simulink model "model_compatible"  (Simulink 7.5)
(part 2 of 2)

  bus2 : powerlib/Measurements/Load Flow Bus  LConnTagsString=a  Phases=single  Connectors=on one side  ID=bus2  Vbase=330000  Vref=1  Vangle=0  VLF=1  VLFb=1  VLFc=1  angleLF=0  angleLFb=0  angleLFc=0
      settings: AttributesFormatString=|
      | %<ID>
      | %<Vbase>V
      | %<VLF>pu
      | %<angleLF>deg.
      | %<Name>
  bus20 : powerlib/Measurements/Load Flow Bus  LConnTagsString=a  Phases=single  Connectors=on one side  ID=bus20  Vbase=330000  Vref=1  Vangle=0  VLF=1  VLFb=1  VLFc=1  angleLF=0  angleLFb=0  angleLFc=0
      settings: AttributesFormatString=|
      | %<ID>
      | %<Vbase>V
      | %<VLF>pu
      | %<angleLF>deg.
      | %<Name>
  bus21 : powerlib/Measurements/Load Flow Bus  LConnTagsString=a  Phases=single  Connectors=on one side  ID=bus21  Vbase=330000  Vref=1  Vangle=0  VLF=1  VLFb=1  VLFc=1  angleLF=0  angleLFb=0  angleLFc=0
      settings: AttributesFormatString=|
      | %<ID>
      | %<Vbase>V
      | %<VLF>pu
      | %<angleLF>deg.
      | %<Name>
  bus22 : powerlib/Measurements/Load Flow Bus  LConnTagsString=a  Phases=single  Connectors=on one side  ID=bus22  Vbase=330000  Vref=1  Vangle=0  VLF=1  VLFb=1  VLFc=1  angleLF=0  angleLFb=0  angleLFc=0
      settings: AttributesFormatString=|
      | %<ID>
      | %<Vbase>V
      | %<VLF>pu
      | %<angleLF>deg.
      | %<Name>
  bus23 : powerlib/Measurements/Load Flow Bus  LConnTagsString=a  Phases=single  Connectors=on one side  ID=bus23  Vbase=330000  Vref=1  Vangle=0  VLF=1  VLFb=1  VLFc=1  angleLF=0  angleLFb=0  angleLFc=0
      settings: AttributesFormatString=|
      | %<ID>
      | %<Vbase>V
      | %<VLF>pu
      | %<angleLF>deg.
      | %<Name>
  bus24 : powerlib/Measurements/Load Flow Bus  LConnTagsString=a  Phases=single  Connectors=on one side  ID=bus24  Vbase=330000  Vref=1  Vangle=0  VLF=1  VLFb=1  VLFc=1  angleLF=0  angleLFb=0  angleLFc=0
      settings: AttributesFormatString=|
      | %<ID>
      | %<Vbase>V
      | %<VLF>pu
      | %<angleLF>deg.
      | %<Name>
  bus25 : powerlib/Measurements/Load Flow Bus  LConnTagsString=a  Phases=single  Connectors=on one side  ID=bus25  Vbase=330000  Vref=1  Vangle=0  VLF=1  VLFb=1  VLFc=1  angleLF=0  angleLFb=0  angleLFc=0
      settings: AttributesFormatString=|
      | %<ID>
      | %<Vbase>V
      | %<VLF>pu
      | %<angleLF>deg.
      | %<Name>
  bus26 : powerlib/Measurements/Load Flow Bus  LConnTagsString=a  Phases=single  Connectors=on one side  ID=bus26  Vbase=330000  Vref=1  Vangle=0  VLF=1  VLFb=1  VLFc=1  angleLF=0  angleLFb=0  angleLFc=0
      settings: AttributesFormatString=|
      | %<ID>
      | %<Vbase>V
      | %<VLF>pu
      | %<angleLF>deg.
      | %<Name>
  bus27 : powerlib/Measurements/Load Flow Bus  LConnTagsString=a  Phases=single  Connectors=on one side  ID=bus27  Vbase=330000  Vref=1  Vangle=0  VLF=1  VLFb=1  VLFc=1  angleLF=0  angleLFb=0  angleLFc=0
      settings: AttributesFormatString=|
      | %<ID>
      | %<Vbase>V
      | %<VLF>pu
      | %<angleLF>deg.
      | %<Name>
  bus28 : powerlib/Measurements/Load Flow Bus  LConnTagsString=a  Phases=single  Connectors=on one side  ID=bus28  Vbase=330000  Vref=1  Vangle=0  VLF=1  VLFb=1  VLFc=1  angleLF=0  angleLFb=0  angleLFc=0
      settings: AttributesFormatString=|
      | %<ID>
      | %<Vbase>V
      | %<VLF>pu
      | %<angleLF>deg.
      | %<Name>
  bus29 : powerlib/Measurements/Load Flow Bus  LConnTagsString=a  Phases=single  Connectors=on one side  ID=bus29  Vbase=330000  Vref=1  Vangle=0  VLF=1  VLFb=1  VLFc=1  angleLF=0  angleLFb=0  angleLFc=0
      settings: AttributesFormatString=|
      | %<ID>
      | %<Vbase>V
      | %<VLF>pu
      | %<angleLF>deg.
      | %<Name>
  bus3 : powerlib/Measurements/Load Flow Bus  LConnTagsString=a  Phases=single  Connectors=on one side  ID=bus3  Vbase=330000  Vref=1  Vangle=0  VLF=1  VLFb=1  VLFc=1  angleLF=0  angleLFb=0  angleLFc=0
      settings: AttributesFormatString=|
      | %<ID>
      | %<Vbase>V
      | %<VLF>pu
      | %<angleLF>deg.
      | %<Name>
  bus30 : powerlib/Measurements/Load Flow Bus  LConnTagsString=a  Phases=single  Connectors=on one side  ID=bus30  Vbase=330000  Vref=1  Vangle=0  VLF=1  VLFb=1  VLFc=1  angleLF=0  angleLFb=0  angleLFc=0
      settings: AttributesFormatString=|
      | %<ID>
      | %<Vbase>V
      | %<VLF>pu
      | %<angleLF>deg.
      | %<Name>
  bus31 : powerlib/Measurements/Load Flow Bus  LConnTagsString=a  Phases=single  Connectors=on one side  ID=bus31  Vbase=330000  Vref=1  Vangle=0  VLF=1  VLFb=1  VLFc=1  angleLF=0  angleLFb=0  angleLFc=0
      settings: AttributesFormatString=|
      | %<ID>
      | %<Vbase>V
      | %<VLF>pu
      | %<angleLF>deg.
      | %<Name>
  bus32 : powerlib/Measurements/Load Flow Bus  LConnTagsString=a  Phases=single  Connectors=on one side  ID=bus32  Vbase=330000  Vref=1  Vangle=0  VLF=1  VLFb=1  VLFc=1  angleLF=0  angleLFb=0  angleLFc=0
      settings: AttributesFormatString=|
      | %<ID>
      | %<Vbase>V
      | %<VLF>pu
      | %<angleLF>deg.
      | %<Name>
  bus33 : powerlib/Measurements/Load Flow Bus  LConnTagsString=a  Phases=single  Connectors=on one side  ID=bus33  Vbase=330000  Vref=1  Vangle=0  VLF=1  VLFb=1  VLFc=1  angleLF=0  angleLFb=0  angleLFc=0
      settings: AttributesFormatString=|
      | %<ID>
      | %<Vbase>V
      | %<VLF>pu
      | %<angleLF>deg.
      | %<Name>
  bus34 : powerlib/Measurements/Load Flow Bus  LConnTagsString=a  Phases=single  Connectors=on one side  ID=bus34  Vbase=330000  Vref=1  Vangle=0  VLF=1  VLFb=1  VLFc=1  angleLF=0  angleLFb=0  angleLFc=0
      settings: AttributesFormatString=|
      | %<ID>
      | %<Vbase>V
      | %<VLF>pu
      | %<angleLF>deg.
      | %<Name>
  bus35 : powerlib/Measurements/Load Flow Bus  LConnTagsString=a  Phases=single  Connectors=on one side  ID=bus35  Vbase=330000  Vref=1  Vangle=0  VLF=1  VLFb=1  VLFc=1  angleLF=0  angleLFb=0  angleLFc=0
      settings: AttributesFormatString=|
      | %<ID>
      | %<Vbase>V
      | %<VLF>pu
      | %<angleLF>deg.
      | %<Name>
  bus36 : powerlib/Measurements/Load Flow Bus  LConnTagsString=a  Phases=single  Connectors=on one side  ID=bus36  Vbase=330000  Vref=1  Vangle=0  VLF=1  VLFb=1  VLFc=1  angleLF=0  angleLFb=0  angleLFc=0
      settings: AttributesFormatString=|
      | %<ID>
      | %<Vbase>V
      | %<VLF>pu
      | %<angleLF>deg.
      | %<Name>
  bus37 : powerlib/Measurements/Load Flow Bus  LConnTagsString=a  Phases=single  Connectors=on one side  ID=bus37  Vbase=330000  Vref=1  Vangle=0  VLF=1  VLFb=1  VLFc=1  angleLF=0  angleLFb=0  angleLFc=0
      settings: AttributesFormatString=|
      | %<ID>
      | %<Vbase>V
      | %<VLF>pu
      | %<angleLF>deg.
      | %<Name>
  bus38 : powerlib/Measurements/Load Flow Bus  LConnTagsString=a  Phases=single  Connectors=on one side  ID=bus38  Vbase=330000  Vref=1  Vangle=0  VLF=1  VLFb=1  VLFc=1  angleLF=0  angleLFb=0  angleLFc=0
      settings: AttributesFormatString=|
      | %<ID>
      | %<Vbase>V
      | %<VLF>pu
      | %<angleLF>deg.
      | %<Name>
  bus39 : powerlib/Measurements/Load Flow Bus  LConnTagsString=a  Phases=single  Connectors=on one side  ID=bus39  Vbase=330000  Vref=1  Vangle=0  VLF=1  VLFb=1  VLFc=1  angleLF=0  angleLFb=0  angleLFc=0
      settings: AttributesFormatString=|
      | %<ID>
      | %<Vbase>V
      | %<VLF>pu
      | %<angleLF>deg.
      | %<Name>
  bus4 : powerlib/Measurements/Load Flow Bus  LConnTagsString=a  Phases=single  Connectors=on one side  ID=bus4  Vbase=330000  Vref=1  Vangle=0  VLF=1  VLFb=1  VLFc=1  angleLF=0  angleLFb=0  angleLFc=0
      settings: AttributesFormatString=|
      | %<ID>
      | %<Vbase>V
      | %<VLF>pu
      | %<angleLF>deg.
      | %<Name>
  bus40 : powerlib/Measurements/Load Flow Bus  LConnTagsString=a  Phases=single  Connectors=on one side  ID=bus40  Vbase=330000  Vref=1  Vangle=0  VLF=1  VLFb=1  VLFc=1  angleLF=0  angleLFb=0  angleLFc=0
      settings: AttributesFormatString=|
      | %<ID>
      | %<Vbase>V
      | %<VLF>pu
      | %<angleLF>deg.
      | %<Name>
  bus41 : powerlib/Measurements/Load Flow Bus  LConnTagsString=a  Phases=single  Connectors=on one side  ID=bus41  Vbase=330000  Vref=1  Vangle=0  VLF=1  VLFb=1  VLFc=1  angleLF=0  angleLFb=0  angleLFc=0
      settings: AttributesFormatString=|
      | %<ID>
      | %<Vbase>V
      | %<VLF>pu
      | %<angleLF>deg.
      | %<Name>
  bus42 : powerlib/Measurements/Load Flow Bus  LConnTagsString=a  Phases=single  Connectors=on one side  ID=bus42  Vbase=330000  Vref=1  Vangle=0  VLF=1  VLFb=1  VLFc=1  angleLF=0  angleLFb=0  angleLFc=0
      settings: AttributesFormatString=|
      | %<ID>
      | %<Vbase>V
      | %<VLF>pu
      | %<angleLF>deg.
      | %<Name>
  bus43 : powerlib/Measurements/Load Flow Bus  LConnTagsString=a  Phases=single  Connectors=on one side  ID=bus43  Vbase=330000  Vref=1  Vangle=0  VLF=1  VLFb=1  VLFc=1  angleLF=0  angleLFb=0  angleLFc=0
      settings: AttributesFormatString=|
      | %<ID>
      | %<Vbase>V
      | %<VLF>pu
      | %<angleLF>deg.
      | %<Name>
  bus44 : powerlib/Measurements/Load Flow Bus  LConnTagsString=a  Phases=single  Connectors=on one side  ID=bus44  Vbase=330000  Vref=1  Vangle=0  VLF=1  VLFb=1  VLFc=1  angleLF=0  angleLFb=0  angleLFc=0
      settings: AttributesFormatString=|
      | %<ID>
      | %<Vbase>V
      | %<VLF>pu
      | %<angleLF>deg.
      | %<Name>
  bus45 : powerlib/Measurements/Load Flow Bus  LConnTagsString=a  Phases=single  Connectors=on one side  ID=bus45  Vbase=330000  Vref=1  Vangle=0  VLF=1  VLFb=1  VLFc=1  angleLF=0  angleLFb=0  angleLFc=0
      settings: AttributesFormatString=|
      | %<ID>
      | %<Vbase>V
      | %<VLF>pu
      | %<angleLF>deg.
      | %<Name>
  bus46 : powerlib/Measurements/Load Flow Bus  LConnTagsString=a  Phases=single  Connectors=on one side  ID=bus46  Vbase=330000  Vref=1  Vangle=0  VLF=1  VLFb=1  VLFc=1  angleLF=0  angleLFb=0  angleLFc=0
      settings: AttributesFormatString=|
      | %<ID>
      | %<Vbase>V
      | %<VLF>pu
      | %<angleLF>deg.
      | %<Name>
  bus47 : powerlib/Measurements/Load Flow Bus  LConnTagsString=a  Phases=single  Connectors=on one side  ID=bus47  Vbase=330000  Vref=1  Vangle=0  VLF=1  VLFb=1  VLFc=1  angleLF=0  angleLFb=0  angleLFc=0
      settings: AttributesFormatString=|
      | %<ID>
      | %<Vbase>V
      | %<VLF>pu
      | %<angleLF>deg.
      | %<Name>
  bus48 : powerlib/Measurements/Load Flow Bus  LConnTagsString=a  Phases=single  Connectors=on one side  ID=bus48  Vbase=330000  Vref=1  Vangle=0  VLF=1  VLFb=1  VLFc=1  angleLF=0  angleLFb=0  angleLFc=0
      settings: AttributesFormatString=|
      | %<ID>
      | %<Vbase>V
      | %<VLF>pu
      | %<angleLF>deg.
      | %<Name>
  bus49 : powerlib/Measurements/Load Flow Bus  LConnTagsString=a  Phases=single  Connectors=on one side  ID=bus49  Vbase=330000  Vref=1  Vangle=0  VLF=1  VLFb=1  VLFc=1  angleLF=0  angleLFb=0  angleLFc=0
      settings: AttributesFormatString=|
      | %<ID>
      | %<Vbase>V
      | %<VLF>pu
      | %<angleLF>deg.
      | %<Name>
  bus5 : powerlib/Measurements/Load Flow Bus  LConnTagsString=a  Phases=single  Connectors=on one side  ID=bus5  Vbase=330000  Vref=1  Vangle=0  VLF=1  VLFb=1  VLFc=1  angleLF=0  angleLFb=0  angleLFc=0
      settings: AttributesFormatString=|
      | %<ID>
      | %<Vbase>V
      | %<VLF>pu
      | %<angleLF>deg.
      | %<Name>
  bus50 : powerlib/Measurements/Load Flow Bus  LConnTagsString=a  Phases=single  Connectors=on one side  ID=bus50  Vbase=330000  Vref=1  Vangle=0  VLF=1  VLFb=1  VLFc=1  angleLF=0  angleLFb=0  angleLFc=0
      settings: AttributesFormatString=|
      | %<ID>
      | %<Vbase>V
      | %<VLF>pu
      | %<angleLF>deg.
      | %<Name>
  bus51 : powerlib/Measurements/Load Flow Bus  LConnTagsString=a  Phases=single  Connectors=on one side  ID=bus51  Vbase=330000  Vref=1  Vangle=0  VLF=1  VLFb=1  VLFc=1  angleLF=0  angleLFb=0  angleLFc=0
      settings: AttributesFormatString=|
      | %<ID>
      | %<Vbase>V
      | %<VLF>pu
      | %<angleLF>deg.
      | %<Name>
  bus52 : powerlib/Measurements/Load Flow Bus  LConnTagsString=a  Phases=single  Connectors=on one side  ID=bus52  Vbase=330000  Vref=1  Vangle=0  VLF=1  VLFb=1  VLFc=1  angleLF=0  angleLFb=0  angleLFc=0
      settings: AttributesFormatString=|
      | %<ID>
      | %<Vbase>V
      | %<VLF>pu
      | %<angleLF>deg.
      | %<Name>
  bus53 : powerlib/Measurements/Load Flow Bus  LConnTagsString=a  Phases=single  Connectors=on one side  ID=bus53  Vbase=330000  Vref=1  Vangle=0  VLF=1  VLFb=1  VLFc=1  angleLF=0  angleLFb=0  angleLFc=0
      settings: AttributesFormatString=|
      | %<ID>
      | %<Vbase>V
      | %<VLF>pu
      | %<angleLF>deg.
      | %<Name>
  bus54 : powerlib/Measurements/Load Flow Bus  LConnTagsString=a  Phases=single  Connectors=on one side  ID=bus54  Vbase=330000  Vref=1  Vangle=0  VLF=1  VLFb=1  VLFc=1  angleLF=0  angleLFb=0  angleLFc=0
      settings: AttributesFormatString=|
      | %<ID>
      | %<Vbase>V
      | %<VLF>pu
      | %<angleLF>deg.
      | %<Name>
  bus55 : powerlib/Measurements/Load Flow Bus  LConnTagsString=a  Phases=single  Connectors=on one side  ID=bus55  Vbase=330000  Vref=1  Vangle=0  VLF=1  VLFb=1  VLFc=1  angleLF=0  angleLFb=0  angleLFc=0
      settings: AttributesFormatString=|
      | %<ID>
      | %<Vbase>V
      | %<VLF>pu
      | %<angleLF>deg.
      | %<Name>
  bus56 : powerlib/Measurements/Load Flow Bus  LConnTagsString=a  Phases=single  Connectors=on one side  ID=bus56  Vbase=330000  Vref=1  Vangle=0  VLF=1  VLFb=1  VLFc=1  angleLF=0  angleLFb=0  angleLFc=0
      settings: AttributesFormatString=|
      | %<ID>
      | %<Vbase>V
      | %<VLF>pu
      | %<angleLF>deg.
      | %<Name>
  bus57 : powerlib/Measurements/Load Flow Bus  LConnTagsString=a  Phases=single  Connectors=on one side  ID=bus57  Vbase=330000  Vref=1  Vangle=0  VLF=1  VLFb=1  VLFc=1  angleLF=0  angleLFb=0  angleLFc=0
      settings: AttributesFormatString=|
      | %<ID>
      | %<Vbase>V
      | %<VLF>pu
      | %<angleLF>deg.
      | %<Name>
  bus58 : powerlib/Measurements/Load Flow Bus  LConnTagsString=a  Phases=single  Connectors=on one side  ID=bus58  Vbase=330000  Vref=1  Vangle=0  VLF=1  VLFb=1  VLFc=1  angleLF=0  angleLFb=0  angleLFc=0
      settings: AttributesFormatString=|
      | %<ID>
      | %<Vbase>V
      | %<VLF>pu
      | %<angleLF>deg.
      | %<Name>
  bus59 : powerlib/Measurements/Load Flow Bus  LConnTagsString=a  Phases=single  Connectors=on one side  ID=bus59  Vbase=330000  Vref=1  Vangle=0  VLF=1  VLFb=1  VLFc=1  angleLF=0  angleLFb=0  angleLFc=0
      settings: AttributesFormatString=|
      | %<ID>
      | %<Vbase>V
      | %<VLF>pu
      | %<angleLF>deg.
      | %<Name>
  bus6 : powerlib/Measurements/Load Flow Bus  LConnTagsString=a  Phases=single  Connectors=on one side  ID=bus6  Vbase=330000  Vref=1  Vangle=0  VLF=1  VLFb=1  VLFc=1  angleLF=0  angleLFb=0  angleLFc=0
      settings: AttributesFormatString=|
      | %<ID>
      | %<Vbase>V
      | %<VLF>pu
      | %<angleLF>deg.
      | %<Name>
  bus60 : powerlib/Measurements/Load Flow Bus  LConnTagsString=a  Phases=single  Connectors=on one side  ID=bus60  Vbase=330000  Vref=1  Vangle=0  VLF=1  VLFb=1  VLFc=1  angleLF=0  angleLFb=0  angleLFc=0
      settings: AttributesFormatString=|
      | %<ID>
      | %<Vbase>V
      | %<VLF>pu
      | %<angleLF>deg.
      | %<Name>
  bus61 : powerlib/Measurements/Load Flow Bus  LConnTagsString=a  Phases=single  Connectors=on one side  ID=bus61  Vbase=330000  Vref=1  Vangle=0  VLF=1  VLFb=1  VLFc=1  angleLF=0  angleLFb=0  angleLFc=0
      settings: AttributesFormatString=|
      | %<ID>
      | %<Vbase>V
      | %<VLF>pu
      | %<angleLF>deg.
      | %<Name>
  bus62 : powerlib/Measurements/Load Flow Bus  LConnTagsString=a  Phases=single  Connectors=on one side  ID=bus62  Vbase=330000  Vref=1  Vangle=0  VLF=1  VLFb=1  VLFc=1  angleLF=0  angleLFb=0  angleLFc=0
      settings: AttributesFormatString=|
      | %<ID>
      | %<Vbase>V
      | %<VLF>pu
      | %<angleLF>deg.
      | %<Name>
  bus63 : powerlib/Measurements/Load Flow Bus  LConnTagsString=a  Phases=single  Connectors=on one side  ID=bus63  Vbase=330000  Vref=1  Vangle=0  VLF=1  VLFb=1  VLFc=1  angleLF=0  angleLFb=0  angleLFc=0
      settings: AttributesFormatString=|
      | %<ID>
      | %<Vbase>V
      | %<VLF>pu
      | %<angleLF>deg.
      | %<Name>
  bus64 : powerlib/Measurements/Load Flow Bus  LConnTagsString=a  Phases=single  Connectors=on one side  ID=bus64  Vbase=330000  Vref=1  Vangle=0  VLF=1  VLFb=1  VLFc=1  angleLF=0  angleLFb=0  angleLFc=0
      settings: AttributesFormatString=|
      | %<ID>
      | %<Vbase>V
      | %<VLF>pu
      | %<angleLF>deg.
      | %<Name>
  bus65 : powerlib/Measurements/Load Flow Bus  LConnTagsString=a  Phases=single  Connectors=on one side  ID=bus65  Vbase=330000  Vref=1  Vangle=0  VLF=1  VLFb=1  VLFc=1  angleLF=0  angleLFb=0  angleLFc=0
      settings: AttributesFormatString=|
      | %<ID>
      | %<Vbase>V
      | %<VLF>pu
      | %<angleLF>deg.
      | %<Name>
  bus66 : powerlib/Measurements/Load Flow Bus  LConnTagsString=a  Phases=single  Connectors=on one side  ID=bus66  Vbase=330000  Vref=1  Vangle=0  VLF=1  VLFb=1  VLFc=1  angleLF=0  angleLFb=0  angleLFc=0
      settings: AttributesFormatString=|
      | %<ID>
      | %<Vbase>V
      | %<VLF>pu
      | %<angleLF>deg.
      | %<Name>
  bus67 : powerlib/Measurements/Load Flow Bus  LConnTagsString=a  Phases=single  Connectors=on one side  ID=bus67  Vbase=330000  Vref=1  Vangle=0  VLF=1  VLFb=1  VLFc=1  angleLF=0  angleLFb=0  angleLFc=0
      settings: AttributesFormatString=|
      | %<ID>
      | %<Vbase>V
      | %<VLF>pu
      | %<angleLF>deg.
      | %<Name>
  bus68 : powerlib/Measurements/Load Flow Bus  LConnTagsString=a  Phases=single  Connectors=on one side  ID=bus68  Vbase=330000  Vref=1  Vangle=0  VLF=1  VLFb=1  VLFc=1  angleLF=0  angleLFb=0  angleLFc=0
      settings: AttributesFormatString=|
      | %<ID>
      | %<Vbase>V
      | %<VLF>pu
      | %<angleLF>deg.
      | %<Name>
  bus69 : powerlib/Measurements/Load Flow Bus  LConnTagsString=a  Phases=single  Connectors=on one side  ID=bus69  Vbase=330000  Vref=1  Vangle=0  VLF=1  VLFb=1  VLFc=1  angleLF=0  angleLFb=0  angleLFc=0
      settings: AttributesFormatString=|
      | %<ID>
      | %<Vbase>V
      | %<VLF>pu
      | %<angleLF>deg.
      | %<Name>
  bus7 : powerlib/Measurements/Load Flow Bus  LConnTagsString=a  Phases=single  Connectors=on one side  ID=bus7  Vbase=330000  Vref=1  Vangle=0  VLF=1  VLFb=1  VLFc=1  angleLF=0  angleLFb=0  angleLFc=0
      settings: AttributesFormatString=|
      | %<ID>
      | %<Vbase>V
      | %<VLF>pu
      | %<angleLF>deg.
      | %<Name>
  bus70 : powerlib/Measurements/Load Flow Bus  LConnTagsString=a  Phases=single  Connectors=on one side  ID=bus70  Vbase=330000  Vref=1  Vangle=0  VLF=1  VLFb=1  VLFc=1  angleLF=0  angleLFb=0  angleLFc=0
      settings: AttributesFormatString=|
      | %<ID>
      | %<Vbase>V
      | %<VLF>pu
      | %<angleLF>deg.
      | %<Name>
  bus71 : powerlib/Measurements/Load Flow Bus  LConnTagsString=a  Phases=single  Connectors=on one side  ID=bus71  Vbase=330000  Vref=1  Vangle=0  VLF=1  VLFb=1  VLFc=1  angleLF=0  angleLFb=0  angleLFc=0
      settings: AttributesFormatString=|
      | %<ID>
      | %<Vbase>V
      | %<VLF>pu
      | %<angleLF>deg.
      | %<Name>
  bus72 : powerlib/Measurements/Load Flow Bus  LConnTagsString=a  Phases=single  Connectors=on one side  ID=bus72  Vbase=330000  Vref=1  Vangle=0  VLF=1  VLFb=1  VLFc=1  angleLF=0  angleLFb=0  angleLFc=0
      settings: AttributesFormatString=|
      | %<ID>
      | %<Vbase>V
      | %<VLF>pu
      | %<angleLF>deg.
      | %<Name>
  bus73 : powerlib/Measurements/Load Flow Bus  LConnTagsString=a  Phases=single  Connectors=on one side  ID=bus73  Vbase=330000  Vref=1  Vangle=0  VLF=1  VLFb=1  VLFc=1  angleLF=0  angleLFb=0  angleLFc=0
      settings: AttributesFormatString=|
      | %<ID>
      | %<Vbase>V
      | %<VLF>pu
      | %<angleLF>deg.
      | %<Name>
  bus74 : powerlib/Measurements/Load Flow Bus  LConnTagsString=a  Phases=single  Connectors=on one side  ID=bus74  Vbase=330000  Vref=1  Vangle=0  VLF=1  VLFb=1  VLFc=1  angleLF=0  angleLFb=0  angleLFc=0
      settings: AttributesFormatString=|
      | %<ID>
      | %<Vbase>V
      | %<VLF>pu
      | %<angleLF>deg.
      | %<Name>
  bus75 : powerlib/Measurements/Load Flow Bus  LConnTagsString=a  Phases=single  Connectors=on one side  ID=bus75  Vbase=330000  Vref=1  Vangle=0  VLF=1  VLFb=1  VLFc=1  angleLF=0  angleLFb=0  angleLFc=0
      settings: AttributesFormatString=|
      | %<ID>
      | %<Vbase>V
      | %<VLF>pu
      | %<angleLF>deg.
      | %<Name>
  bus76 : powerlib/Measurements/Load Flow Bus  LConnTagsString=a  Phases=single  Connectors=on one side  ID=bus76  Vbase=330000  Vref=1  Vangle=0  VLF=1  VLFb=1  VLFc=1  angleLF=0  angleLFb=0  angleLFc=0
      settings: AttributesFormatString=|
      | %<ID>
      | %<Vbase>V
      | %<VLF>pu
      | %<angleLF>deg.
      | %<Name>
  bus77 : powerlib/Measurements/Load Flow Bus  LConnTagsString=a  Phases=single  Connectors=on one side  ID=bus77  Vbase=330000  Vref=1  Vangle=0  VLF=1  VLFb=1  VLFc=1  angleLF=0  angleLFb=0  angleLFc=0
      settings: AttributesFormatString=|
      | %<ID>
      | %<Vbase>V
      | %<VLF>pu
      | %<angleLF>deg.
      | %<Name>
  bus78 : powerlib/Measurements/Load Flow Bus  LConnTagsString=a  Phases=single  Connectors=on one side  ID=bus78  Vbase=330000  Vref=1  Vangle=0  VLF=1  VLFb=1  VLFc=1  angleLF=0  angleLFb=0  angleLFc=0
      settings: AttributesFormatString=|
      | %<ID>
      | %<Vbase>V
      | %<VLF>pu
      | %<angleLF>deg.
      | %<Name>
  bus79 : powerlib/Measurements/Load Flow Bus  LConnTagsString=a  Phases=single  Connectors=on one side  ID=bus79  Vbase=10000  Vref=1  Vangle=0  VLF=1  VLFb=1  VLFc=1  angleLF=0  angleLFb=0  angleLFc=0
      settings: AttributesFormatString=|
      | %<ID>
      | %<Vbase>V
      | %<VLF>pu
      | %<angleLF>deg.
      | %<Name>
  bus8 : powerlib/Measurements/Load Flow Bus  LConnTagsString=a  Phases=single  Connectors=on one side  ID=bus8  Vbase=330000  Vref=1  Vangle=0  VLF=1  VLFb=1  VLFc=1  angleLF=0  angleLFb=0  angleLFc=0
      settings: AttributesFormatString=|
      | %<ID>
      | %<Vbase>V
      | %<VLF>pu
      | %<angleLF>deg.
      | %<Name>
  bus80 : powerlib/Measurements/Load Flow Bus  LConnTagsString=a  Phases=single  Connectors=on one side  ID=bus80  Vbase=10000  Vref=1  Vangle=0  VLF=1  VLFb=1  VLFc=1  angleLF=0  angleLFb=0  angleLFc=0
      settings: AttributesFormatString=|
      | %<ID>
      | %<Vbase>V
      | %<VLF>pu
      | %<angleLF>deg.
      | %<Name>
  bus81 : powerlib/Measurements/Load Flow Bus  LConnTagsString=a  Phases=single  Connectors=on one side  ID=bus81  Vbase=6000  Vref=1  Vangle=0  VLF=1  VLFb=1  VLFc=1  angleLF=0  angleLFb=0  angleLFc=0
      settings: AttributesFormatString=|
      | %<ID>
      | %<Vbase>V
      | %<VLF>pu
      | %<angleLF>deg.
      | %<Name>
  bus82 : powerlib/Measurements/Load Flow Bus  LConnTagsString=a  Phases=single  Connectors=on one side  ID=bus82  Vbase=330000  Vref=1  Vangle=0  VLF=1  VLFb=1  VLFc=1  angleLF=0  angleLFb=0  angleLFc=0
      settings: AttributesFormatString=|
      | %<ID>
      | %<Vbase>V
      | %<VLF>pu
      | %<angleLF>deg.
      | %<Name>
  bus83 : powerlib/Measurements/Load Flow Bus  LConnTagsString=a  Phases=single  Connectors=on one side  ID=bus83  Vbase=330000  Vref=1  Vangle=0  VLF=1  VLFb=1  VLFc=1  angleLF=0  angleLFb=0  angleLFc=0
      settings: AttributesFormatString=|
      | %<ID>
      | %<Vbase>V
      | %<VLF>pu
      | %<angleLF>deg.
      | %<Name>
  bus84 : powerlib/Measurements/Load Flow Bus  LConnTagsString=a  Phases=single  Connectors=on one side  ID=bus84  Vbase=330000  Vref=1  Vangle=0  VLF=1  VLFb=1  VLFc=1  angleLF=0  angleLFb=0  angleLFc=0
      settings: AttributesFormatString=|
      | %<ID>
      | %<Vbase>V
      | %<VLF>pu
      | %<angleLF>deg.
      | %<Name>
  bus85 : powerlib/Measurements/Load Flow Bus  LConnTagsString=a  Phases=single  Connectors=on one side  ID=bus85  Vbase=330000  Vref=1  Vangle=0  VLF=1  VLFb=1  VLFc=1  angleLF=0  angleLFb=0  angleLFc=0
      settings: AttributesFormatString=|
      | %<ID>
      | %<Vbase>V
      | %<VLF>pu
      | %<angleLF>deg.
      | %<Name>
  bus86 : powerlib/Measurements/Load Flow Bus  LConnTagsString=a  Phases=single  Connectors=on one side  ID=bus86  Vbase=35000  Vref=1  Vangle=0  VLF=1  VLFb=1  VLFc=1  angleLF=0  angleLFb=0  angleLFc=0
      settings: AttributesFormatString=|
      | %<ID>
      | %<Vbase>V
      | %<VLF>pu
      | %<angleLF>deg.
      | %<Name>
  bus87 : powerlib/Measurements/Load Flow Bus  LConnTagsString=a  Phases=single  Connectors=on one side  ID=bus87  Vbase=15000  Vref=1  Vangle=0  VLF=1  VLFb=1  VLFc=1  angleLF=0  angleLFb=0  angleLFc=0
      settings: AttributesFormatString=|
      | %<ID>
      | %<Vbase>V
      | %<VLF>pu
      | %<angleLF>deg.
      | %<Name>
  bus88 : powerlib/Measurements/Load Flow Bus  LConnTagsString=a  Phases=single  Connectors=on one side  ID=bus88  Vbase=10000  Vref=1  Vangle=0  VLF=1  VLFb=1  VLFc=1  angleLF=0  angleLFb=0  angleLFc=0
      settings: AttributesFormatString=|
      | %<ID>
      | %<Vbase>V
      | %<VLF>pu
      | %<angleLF>deg.
      | %<Name>
  bus89 : powerlib/Measurements/Load Flow Bus  LConnTagsString=a  Phases=single  Connectors=on one side  ID=bus89  Vbase=10000  Vref=1  Vangle=0  VLF=1  VLFb=1  VLFc=1  angleLF=0  angleLFb=0  angleLFc=0
      settings: AttributesFormatString=|
      | %<ID>
      | %<Vbase>V
      | %<VLF>pu
      | %<angleLF>deg.
      | %<Name>
  bus9 : powerlib/Measurements/Load Flow Bus  LConnTagsString=a  Phases=single  Connectors=on one side  ID=bus9  Vbase=330000  Vref=1  Vangle=0  VLF=1  VLFb=1  VLFc=1  angleLF=0  angleLFb=0  angleLFc=0
      settings: AttributesFormatString=|
      | %<ID>
      | %<Vbase>V
      | %<VLF>pu
      | %<angleLF>deg.
      | %<Name>
  bus90 : powerlib/Measurements/Load Flow Bus  LConnTagsString=a  Phases=single  Connectors=on one side  ID=bus90  Vbase=110000  Vref=1  Vangle=0  VLF=1  VLFb=1  VLFc=1  angleLF=0  angleLFb=0  angleLFc=0
      settings: AttributesFormatString=|
      | %<ID>
      | %<Vbase>V
      | %<VLF>pu
      | %<angleLF>deg.
      | %<Name>
  bus91 : powerlib/Measurements/Load Flow Bus  LConnTagsString=a  Phases=single  Connectors=on one side  ID=bus91  Vbase=35000  Vref=1  Vangle=0  VLF=1  VLFb=1  VLFc=1  angleLF=0  angleLFb=0  angleLFc=0
      settings: AttributesFormatString=|
      | %<ID>
      | %<Vbase>V
      | %<VLF>pu
      | %<angleLF>deg.
      | %<Name>
  bus92 : powerlib/Measurements/Load Flow Bus  LConnTagsString=a  Phases=single  Connectors=on one side  ID=bus92  Vbase=10000  Vref=1  Vangle=0  VLF=1  VLFb=1  VLFc=1  angleLF=0  angleLFb=0  angleLFc=0
      settings: AttributesFormatString=|
      | %<ID>
      | %<Vbase>V
      | %<VLF>pu
      | %<angleLF>deg.
      | %<Name>
  bus93 : powerlib/Measurements/Load Flow Bus  LConnTagsString=a  Phases=single  Connectors=on one side  ID=bus93  Vbase=15000  Vref=1  Vangle=0  VLF=1  VLFb=1  VLFc=1  angleLF=0  angleLFb=0  angleLFc=0
      settings: AttributesFormatString=|
      | %<ID>
      | %<Vbase>V
      | %<VLF>pu
      | %<angleLF>deg.
      | %<Name>
  bus94 : powerlib/Measurements/Load Flow Bus  LConnTagsString=a  Phases=single  Connectors=on one side  ID=bus94  Vbase=330000  Vref=1  Vangle=0  VLF=1  VLFb=1  VLFc=1  angleLF=0  angleLFb=0  angleLFc=0
      settings: AttributesFormatString=|
      | %<ID>
      | %<Vbase>V
      | %<VLF>pu
      | %<angleLF>deg.
      | %<Name>
  bus95 : powerlib/Measurements/Load Flow Bus  LConnTagsString=a  Phases=single  Connectors=on one side  ID=bus95  Vbase=10000  Vref=1  Vangle=0  VLF=1  VLFb=1  VLFc=1  angleLF=0  angleLFb=0  angleLFc=0
      settings: AttributesFormatString=|
      | %<ID>
      | %<Vbase>V
      | %<VLF>pu
      | %<angleLF>deg.
      | %<Name>
  bus96 : powerlib/Measurements/Load Flow Bus  LConnTagsString=a  Phases=single  Connectors=on one side  ID=bus96  Vbase=330000  Vref=1  Vangle=0  VLF=1  VLFb=1  VLFc=1  angleLF=0  angleLFb=0  angleLFc=0
      settings: AttributesFormatString=|
      | %<ID>
      | %<Vbase>V
      | %<VLF>pu
      | %<angleLF>deg.
      | %<Name>
  bus97 : powerlib/Measurements/Load Flow Bus  LConnTagsString=a  Phases=single  Connectors=on one side  ID=bus97  Vbase=330000  Vref=1  Vangle=0  VLF=1  VLFb=1  VLFc=1  angleLF=0  angleLFb=0  angleLFc=0
      settings: AttributesFormatString=|
      | %<ID>
      | %<Vbase>V
      | %<VLF>pu
      | %<angleLF>deg.
      | %<Name>
  bus98 : powerlib/Measurements/Load Flow Bus  LConnTagsString=a  Phases=single  Connectors=on one side  ID=bus98  Vbase=330000  Vref=1  Vangle=0  VLF=1  VLFb=1  VLFc=1  angleLF=0  angleLFb=0  angleLFc=0
      settings: AttributesFormatString=|
      | %<ID>
      | %<Vbase>V
      | %<VLF>pu
      | %<angleLF>deg.
      | %<Name>
  bus99 : powerlib/Measurements/Load Flow Bus  LConnTagsString=a  Phases=single  Connectors=on one side  ID=bus99  Vbase=330000  Vref=1  Vangle=0  VLF=1  VLFb=1  VLFc=1  angleLF=0  angleLFb=0  angleLFc=0
      settings: AttributesFormatString=|
      | %<ID>
      | %<Vbase>V
      | %<VLF>pu
      | %<angleLF>deg.
      | %<Name>
  powergui : powerlib/powergui  Priority=1  SimulationMode=Phasor  SolverType=Tustin/Backward Euler (TBE)  SampleTime=50e-6  frequency=50  SPID=off  DisableSnubberDevices=off  DisableRonSwitches=off  DisableVfSwitches=off  SwTol=0  DisplayEquations=off  Interpol=off  ExternalGateDelay=off  methode=off  Ts=10  FunctionMessages=off  echomessages=off  HookPort=off  EnableUseOfTLC=off  x0status=blocks  frequencyindice=50  Pbase=3000e6  ErrMax=0.0001  Iterations=50  UnitsV=V  UnitsW=W  buscounter=0  RestoreLinks=warning  ResistiveCurrentMeasurement=off  Frange=[0:2:500]  Ylog=off  Xlog=on  ShowGrid=off  save=off  variable=ZData  structure=0  ZoomFFT=off  StartTime=0.0  cycles=1  DisplayStyle=1  fundamental=60  FreqAxis=off  MaxFrequency=1000  frequencyindicesteady=1  RmsSteady=1  display=off
  connections:
  _CN_182915221_330000_CN182796002/LConn1 -- T_182915221_330000;110000;10000_Харцизька_330/LConn1 -- _CN_182915221_330000_CN_165762303_330000/LConn1 -- _CN_182915221_330000_CN_259021748_330000/LConn1
  _CN_182915221_330000_CN182796002/LConn2 -- T_182915221_330000;110000;10000_Харцизька_330/LConn2 -- _CN_182915221_330000_CN_165762303_330000/LConn2 -- _CN_182915221_330000_CN_259021748_330000/LConn2
  _CN_182915221_330000_CN182796002/LConn3 -- T_182915221_330000;110000;10000_Харцизька_330/LConn3 -- _CN_182915221_330000_CN_165762303_330000/LConn3 -- bus1/LConn1 -- _CN_182915221_330000_CN_259021748_330000/LConn3
  G_182796002_Зуевская_ТЭС/RConn1 -- _CN_182915221_330000_CN182796002/RConn1
  G_182796002_Зуевская_ТЭС/RConn2 -- _CN_182915221_330000_CN182796002/RConn2
  _CN_182915221_330000_CN182796002/RConn3 -- G_182796002_Зуевская_ТЭС/RConn3 -- bus2/LConn1
  _CN_182915221_330000_CN_259021748_330000/RConn1 -- T_259021748_330000;110000;10000_Зоря_330/LConn1 -- _CN_296751070_330000_CN_259021748_330000/LConn1 -- _CN_172507826_330000_CN_259021748_330000/LConn1 -- _CN_289148613_330000_CN_259021748_330000/LConn1
  _CN_182915221_330000_CN_259021748_330000/RConn2 -- T_259021748_330000;110000;10000_Зоря_330/LConn2 -- _CN_296751070_330000_CN_259021748_330000/LConn2 -- _CN_172507826_330000_CN_259021748_330000/LConn2 -- _CN_289148613_330000_CN_259021748_330000/LConn2
  _CN_182915221_330000_CN_259021748_330000/RConn3 -- T_259021748_330000;110000;10000_Зоря_330/LConn3 -- _CN_296751070_330000_CN_259021748_330000/LConn3 -- _CN_172507826_330000_CN_259021748_330000/LConn3 -- _CN_289148613_330000_CN_259021748_330000/LConn3 -- bus3/LConn1
  _CN_182915221_330000_CN_165762303_330000/RConn1 -- T_165762303_330000;220000;110000;35000;6000_Чайкіне_330/LConn1 -- _CN_296751070_330000_CN_165762303_330000/LConn1
  _CN_182915221_330000_CN_165762303_330000/RConn2 -- T_165762303_330000;220000;110000;35000;6000_Чайкіне_330/LConn2 -- _CN_296751070_330000_CN_165762303_330000/LConn2
  _CN_182915221_330000_CN_165762303_330000/RConn3 -- T_165762303_330000;220000;110000;35000;6000_Чайкіне_330/LConn3 -- _CN_296751070_330000_CN_165762303_330000/LConn3 -- bus4/LConn1
  T_155861889__/LConn1 -- _CN_155861889_330000_CN_155861891_330000/LConn1
  T_155861889__/LConn2 -- _CN_155861889_330000_CN_155861891_330000/LConn2
  _CN_155861889_330000_CN_155861891_330000/LConn3 -- T_155861889__/LConn3 -- bus5/LConn1
  _CN_155861889_330000_CN_155861891_330000/RConn1 -- T_155861891__/LConn1 -- _CN_155861891_330000_CN_274598688_330000/LConn1
  _CN_155861889_330000_CN_155861891_330000/RConn2 -- T_155861891__/LConn2 -- _CN_155861891_330000_CN_274598688_330000/LConn2
  _CN_155861889_330000_CN_155861891_330000/RConn3 -- T_155861891__/LConn3 -- _CN_155861891_330000_CN_274598688_330000/LConn3 -- bus6/LConn1
  _CN_155861891_330000_CN_274598688_330000/RConn1 -- T_274598688__Аджалик_330/LConn1 -- _CN_274598688_330000_CN_28878309_330000/LConn1 -- _CN_274598688_330000_CN_296496011_330000/LConn1
  _CN_155861891_330000_CN_274598688_330000/RConn2 -- T_274598688__Аджалик_330/LConn2 -- _CN_274598688_330000_CN_28878309_330000/LConn2 -- _CN_274598688_330000_CN_296496011_330000/LConn2
  _CN_155861891_330000_CN_274598688_330000/RConn3 -- T_274598688__Аджалик_330/LConn3 -- _CN_274598688_330000_CN_28878309_330000/LConn3 -- _CN_274598688_330000_CN_296496011_330000/LConn3 -- bus7/LConn1
  _CN_292523027_330000_CN_135644235_330000/LConn1 -- T_292523027__/LConn1 -- _CN_292523027_330000_CN_219508915_330000/LConn1 -- _CN_292523027_330000_CN_188001625_330000/LConn1 -- _CN_292523027_330000_CN132697290/LConn1 -- _CN_292523027_330000_CN_176443878_330000/LConn1
  _CN_292523027_330000_CN_135644235_330000/LConn2 -- T_292523027__/LConn2 -- _CN_292523027_330000_CN_219508915_330000/LConn2 -- _CN_292523027_330000_CN_188001625_330000/LConn2 -- _CN_292523027_330000_CN132697290/LConn2 -- _CN_292523027_330000_CN_176443878_330000/LConn2
  _CN_292523027_330000_CN_135644235_330000/LConn3 -- T_292523027__/LConn3 -- _CN_292523027_330000_CN_219508915_330000/LConn3 -- _CN_292523027_330000_CN_188001625_330000/LConn3 -- _CN_292523027_330000_CN132697290/LConn3 -- _CN_292523027_330000_CN_176443878_330000/LConn3 -- bus8/LConn1
  T_135644235_400000;330000;220000;110000;35000_Михайлівка_330/LConn1 -- _CN_292523027_330000_CN_135644235_330000/RConn1
  T_135644235_400000;330000;220000;110000;35000_Михайлівка_330/LConn2 -- _CN_292523027_330000_CN_135644235_330000/RConn2
  _CN_292523027_330000_CN_135644235_330000/RConn3 -- T_135644235_400000;330000;220000;110000;35000_Михайлівка_330/LConn3 -- bus9/LConn1
  _CN_292523027_330000_CN_219508915_330000/RConn1 -- T_219508915_750000;500000;330000;15000_Донбаська_750/LConn1 -- _CN_130513926_330000_CN_219508915_330000/LConn1
  _CN_292523027_330000_CN_219508915_330000/RConn2 -- T_219508915_750000;500000;330000;15000_Донбаська_750/LConn2 -- _CN_130513926_330000_CN_219508915_330000/LConn2
  _CN_292523027_330000_CN_219508915_330000/RConn3 -- T_219508915_750000;500000;330000;15000_Донбаська_750/LConn3 -- _CN_130513926_330000_CN_219508915_330000/LConn3 -- bus10/LConn1
  _CN_292523027_330000_CN_188001625_330000/RConn1 -- T_188001625_330000;110000;35000;10000_«Центральна»_330_110_35_кВ/LConn1 -- _CN_292523016_330000_CN_188001625_330000/LConn1 -- _CN_130513926_330000_CN_188001625_330000/LConn1 -- _CN_171816615_330000_CN_188001625_330000/LConn1
  _CN_292523027_330000_CN_188001625_330000/RConn2 -- T_188001625_330000;110000;35000;10000_«Центральна»_330_110_35_кВ/LConn2 -- _CN_292523016_330000_CN_188001625_330000/LConn2 -- _CN_130513926_330000_CN_188001625_330000/LConn2 -- _CN_171816615_330000_CN_188001625_330000/LConn2
  _CN_292523027_330000_CN_188001625_330000/RConn3 -- T_188001625_330000;110000;35000;10000_«Центральна»_330_110_35_кВ/LConn3 -- _CN_292523016_330000_CN_188001625_330000/LConn3 -- _CN_130513926_330000_CN_188001625_330000/LConn3 -- _CN_171816615_330000_CN_188001625_330000/LConn3 -- bus11/LConn1
  G_132697290_Вуглегірська_ТЕС/RConn1 -- _CN_292523027_330000_CN132697290/RConn1
  G_132697290_Вуглегірська_ТЕС/RConn2 -- _CN_292523027_330000_CN132697290/RConn2
  _CN_292523027_330000_CN132697290/RConn3 -- G_132697290_Вуглегірська_ТЕС/RConn3 -- bus12/LConn1
  _CN_292523027_330000_CN_176443878_330000/RConn1 -- T_176443878_330000;110000;35000;10000_Макіївська/LConn1 -- _CN_296751070_330000_CN_176443878_330000/LConn1
  _CN_292523027_330000_CN_176443878_330000/RConn2 -- T_176443878_330000;110000;35000;10000_Макіївська/LConn2 -- _CN_296751070_330000_CN_176443878_330000/LConn2
  _CN_292523027_330000_CN_176443878_330000/RConn3 -- T_176443878_330000;110000;35000;10000_Макіївська/LConn3 -- _CN_296751070_330000_CN_176443878_330000/LConn3 -- bus13/LConn1
  "T_99234566_330000;110000_ПС_330_110_кВ_\"Білоцерківська\""/LConn1 -- _CN_99234566_330000_CN_211109125_330000/LConn1
  "T_99234566_330000;110000_ПС_330_110_кВ_\"Білоцерківська\""/LConn2 -- _CN_99234566_330000_CN_211109125_330000/LConn2
  _CN_99234566_330000_CN_211109125_330000/LConn3 -- "T_99234566_330000;110000_ПС_330_110_кВ_\"Білоцерківська\""/LConn3 -- bus14/LConn1
  _CN_99234566_330000_CN_211109125_330000/RConn1 -- T_211109125_330000;110000;35000_Козятин_330/LConn1 -- _CN_70994591_330000_CN_211109125_330000/LConn1
  _CN_99234566_330000_CN_211109125_330000/RConn2 -- T_211109125_330000;110000;35000_Козятин_330/LConn2 -- _CN_70994591_330000_CN_211109125_330000/LConn2
  _CN_99234566_330000_CN_211109125_330000/RConn3 -- T_211109125_330000;110000;35000_Козятин_330/LConn3 -- _CN_70994591_330000_CN_211109125_330000/LConn3 -- bus15/LConn1
  T_157927169_330000;150000;10000_ПС_Дніпропетровська_330/LConn1 -- _CN_157927169_330000_CN_209879378_330000/LConn1
  T_157927169_330000;150000;10000_ПС_Дніпропетровська_330/LConn2 -- _CN_157927169_330000_CN_209879378_330000/LConn2
  _CN_157927169_330000_CN_209879378_330000/LConn3 -- T_157927169_330000;150000;10000_ПС_Дніпропетровська_330/LConn3 -- bus16/LConn1
  _CN_157927169_330000_CN_209879378_330000/RConn1 -- T_209879378_750000;330000;35000;15000_Запорізька_750/LConn1 -- _CN_209879378_330000_CN281269420/LConn1
  _CN_157927169_330000_CN_209879378_330000/RConn2 -- T_209879378_750000;330000;35000;15000_Запорізька_750/LConn2 -- _CN_209879378_330000_CN281269420/LConn2
  _CN_157927169_330000_CN_209879378_330000/RConn3 -- T_209879378_750000;330000;35000;15000_Запорізька_750/LConn3 -- _CN_209879378_330000_CN281269420/LConn3 -- bus17/LConn1
  _CN_292523016_330000_CN_188001625_330000/RConn1 -- T_292523016__Лозова/LConn1 -- _CN_292523016_330000_CN_203926610_330000/LConn1
  _CN_292523016_330000_CN_188001625_330000/RConn2 -- T_292523016__Лозова/LConn2 -- _CN_292523016_330000_CN_203926610_330000/LConn2
  _CN_292523016_330000_CN_188001625_330000/RConn3 -- T_292523016__Лозова/LConn3 -- _CN_292523016_330000_CN_203926610_330000/LConn3 -- bus18/LConn1
  _CN_292523016_330000_CN_203926610_330000/RConn1 -- T_203926610_330000;110000;10000_Первомайськ_330/LConn1 -- _CN_215079308_330000_CN_203926610_330000/LConn1 -- _CN_203926610_330000_CN272744229/LConn1
  _CN_292523016_330000_CN_203926610_330000/RConn2 -- T_203926610_330000;110000;10000_Первомайськ_330/LConn2 -- _CN_215079308_330000_CN_203926610_330000/LConn2 -- _CN_203926610_330000_CN272744229/LConn2
  _CN_292523016_330000_CN_203926610_330000/RConn3 -- T_203926610_330000;110000;10000_Первомайськ_330/LConn3 -- _CN_215079308_330000_CN_203926610_330000/LConn3 -- _CN_203926610_330000_CN272744229/LConn3 -- bus19/LConn1
  _CN_104864777_330000_CN_237532980_330000/LConn1 -- T_104864777__/LConn1 -- _CN_104864777_330000_CN_168587285_330000/LConn1
  _CN_104864777_330000_CN_237532980_330000/LConn2 -- T_104864777__/LConn2 -- _CN_104864777_330000_CN_168587285_330000/LConn2
  _CN_104864777_330000_CN_237532980_330000/LConn3 -- T_104864777__/LConn3 -- _CN_104864777_330000_CN_168587285_330000/LConn3 -- bus20/LConn1
  _CN_104864777_330000_CN_237532980_330000/RConn1 -- T_237532980__/LConn1 -- _CN_237532980_330000_CN_159727866_330000/LConn1
  _CN_104864777_330000_CN_237532980_330000/RConn2 -- T_237532980__/LConn2 -- _CN_237532980_330000_CN_159727866_330000/LConn2
  _CN_104864777_330000_CN_237532980_330000/RConn3 -- T_237532980__/LConn3 -- _CN_237532980_330000_CN_159727866_330000/LConn3 -- bus21/LConn1
  _CN_104864777_330000_CN_168587285_330000/RConn1 -- T_168587285__/LConn1 -- _CN_168587285_330000_CN_116452049_330000/LConn1
  _CN_104864777_330000_CN_168587285_330000/RConn2 -- T_168587285__/LConn2 -- _CN_168587285_330000_CN_116452049_330000/LConn2
  _CN_104864777_330000_CN_168587285_330000/RConn3 -- T_168587285__/LConn3 -- _CN_168587285_330000_CN_116452049_330000/LConn3 -- bus22/LConn1
  _CN_74481802_330000_CN_70994591_330000/LConn1 -- T_74481802__Вінниця_330/LConn1 -- _CN_74481802_330000_CN_212379146_330000/LConn1
  _CN_74481802_330000_CN_70994591_330000/LConn2 -- T_74481802__Вінниця_330/LConn2 -- _CN_74481802_330000_CN_212379146_330000/LConn2
  _CN_74481802_330000_CN_70994591_330000/LConn3 -- T_74481802__Вінниця_330/LConn3 -- _CN_74481802_330000_CN_212379146_330000/LConn3 -- bus23/LConn1
  _CN_74481802_330000_CN_70994591_330000/RConn1 -- T_70994591_750000;330000;110000_Вінниця_750/LConn1 -- _CN_70994591_330000_CN_211109125_330000/RConn1
  _CN_74481802_330000_CN_70994591_330000/RConn2 -- T_70994591_750000;330000;110000_Вінниця_750/LConn2 -- _CN_70994591_330000_CN_211109125_330000/RConn2
  _CN_74481802_330000_CN_70994591_330000/RConn3 -- T_70994591_750000;330000;110000_Вінниця_750/LConn3 -- _CN_70994591_330000_CN_211109125_330000/RConn3 -- bus24/LConn1
  T_212379146__Бар_330/LConn1 -- _CN_74481802_330000_CN_212379146_330000/RConn1
  T_212379146__Бар_330/LConn2 -- _CN_74481802_330000_CN_212379146_330000/RConn2
  _CN_74481802_330000_CN_212379146_330000/RConn3 -- T_212379146__Бар_330/LConn3 -- bus25/LConn1
  "T_169821963_330000_ПС_330_кВ_\"Чернівці\""/LConn1 -- _CN_169821963_330000_CN_275503522_330000/LConn1
  "T_169821963_330000_ПС_330_кВ_\"Чернівці\""/LConn2 -- _CN_169821963_330000_CN_275503522_330000/LConn2
  _CN_169821963_330000_CN_275503522_330000/LConn3 -- "T_169821963_330000_ПС_330_кВ_\"Чернівці\""/LConn3 -- bus26/LConn1
  T_275503522__Кам’янець_Подільська_330/LConn1 -- _CN_169821963_330000_CN_275503522_330000/RConn1
  T_275503522__Кам’янець_Подільська_330/LConn2 -- _CN_169821963_330000_CN_275503522_330000/RConn2
  _CN_169821963_330000_CN_275503522_330000/RConn3 -- T_275503522__Кам’янець_Подільська_330/LConn3 -- bus27/LConn1
  _CN_215079308_330000_CN_269056567_330000/LConn1 -- "T_215079308_330000_Підстанція_\"Полтава\""/LConn1 -- _CN_215079308_330000_CN_203926610_330000/RConn1 -- _CN_215079308_330000_CN272744229/LConn1 -- _CN_215079308_330000_CN_211101137_330000/LConn1 -- _CN_215079308_330000_CN_294742933_330000/LConn1
  _CN_215079308_330000_CN_269056567_330000/LConn2 -- "T_215079308_330000_Підстанція_\"Полтава\""/LConn2 -- _CN_215079308_330000_CN_203926610_330000/RConn2 -- _CN_215079308_330000_CN272744229/LConn2 -- _CN_215079308_330000_CN_211101137_330000/LConn2 -- _CN_215079308_330000_CN_294742933_330000/LConn2
  _CN_215079308_330000_CN_269056567_330000/LConn3 -- "T_215079308_330000_Підстанція_\"Полтава\""/LConn3 -- _CN_215079308_330000_CN_203926610_330000/RConn3 -- _CN_215079308_330000_CN272744229/LConn3 -- _CN_215079308_330000_CN_211101137_330000/LConn3 -- bus28/LConn1 -- _CN_215079308_330000_CN_294742933_330000/LConn3
  "T_269056567_330000_ПС_330_154_35_10_кВ_\"Кременчук\""/LConn1 -- _CN_215079308_330000_CN_269056567_330000/RConn1
  "T_269056567_330000_ПС_330_154_35_10_кВ_\"Кременчук\""/LConn2 -- _CN_215079308_330000_CN_269056567_330000/RConn2
  _CN_215079308_330000_CN_269056567_330000/RConn3 -- "T_269056567_330000_ПС_330_154_35_10_кВ_\"Кременчук\""/LConn3 -- bus29/LConn1
  _CN_215079308_330000_CN_294742933_330000/RConn1 -- T_294742933__Миргород_330/LConn1 -- _CN_294742933_330000_CN_211101137_330000/LConn1
  _CN_215079308_330000_CN_294742933_330000/RConn2 -- T_294742933__Миргород_330/LConn2 -- _CN_294742933_330000_CN_211101137_330000/LConn2
  _CN_215079308_330000_CN_294742933_330000/RConn3 -- T_294742933__Миргород_330/LConn3 -- _CN_294742933_330000_CN_211101137_330000/LConn3 -- bus30/LConn1
  _CN_215079308_330000_CN272744229/RConn1 -- G_272744229_Зміївська_ТЕС/RConn1 -- _CN_203926610_330000_CN272744229/RConn1
  _CN_215079308_330000_CN272744229/RConn2 -- G_272744229_Зміївська_ТЕС/RConn2 -- _CN_203926610_330000_CN272744229/RConn2
  _CN_215079308_330000_CN272744229/RConn3 -- G_272744229_Зміївська_ТЕС/RConn3 -- _CN_203926610_330000_CN272744229/RConn3 -- bus31/LConn1
  _CN_215079308_330000_CN_211101137_330000/RConn1 -- T_211101137__Північноукраїнська_750/LConn1 -- _CN_236724724_330000_CN_211101137_330000/LConn1 -- _CN_294742933_330000_CN_211101137_330000/RConn1
  _CN_215079308_330000_CN_211101137_330000/RConn2 -- T_211101137__Північноукраїнська_750/LConn2 -- _CN_236724724_330000_CN_211101137_330000/LConn2 -- _CN_294742933_330000_CN_211101137_330000/RConn2
  _CN_215079308_330000_CN_211101137_330000/RConn3 -- T_211101137__Північноукраїнська_750/LConn3 -- _CN_236724724_330000_CN_211101137_330000/LConn3 -- _CN_294742933_330000_CN_211101137_330000/RConn3 -- bus32/LConn1
  _CN_274597272_330000_CN_269527797_330000/LConn1 -- T_274597272_330000;150000;35000_Херсонська_330/LConn1 -- _CN_274597272_330000_CN_221427829_330000/LConn1
  _CN_274597272_330000_CN_269527797_330000/LConn2 -- T_274597272_330000;150000;35000_Херсонська_330/LConn2 -- _CN_274597272_330000_CN_221427829_330000/LConn2
  _CN_274597272_330000_CN_269527797_330000/LConn3 -- T_274597272_330000;150000;35000_Херсонська_330/LConn3 -- _CN_274597272_330000_CN_221427829_330000/LConn3 -- bus33/LConn1
  _CN_274597272_330000_CN_269527797_330000/RConn1 -- "T_269527797_330000;220000;154000;35000;6000_ПС_330_220_150_кВ_\"Новокаховська\""/LConn1 -- _CN_269527797_330000_CN_123451079_330000/LConn1 -- _CN_269527797_330000_CN_97576344_330000/LConn1
  _CN_274597272_330000_CN_269527797_330000/RConn2 -- "T_269527797_330000;220000;154000;35000;6000_ПС_330_220_150_кВ_\"Новокаховська\""/LConn2 -- _CN_269527797_330000_CN_123451079_330000/LConn2 -- _CN_269527797_330000_CN_97576344_330000/LConn2
  _CN_274597272_330000_CN_269527797_330000/RConn3 -- "T_269527797_330000;220000;154000;35000;6000_ПС_330_220_150_кВ_\"Новокаховська\""/LConn3 -- _CN_269527797_330000_CN_123451079_330000/LConn3 -- bus34/LConn1 -- _CN_269527797_330000_CN_97576344_330000/LConn3
  T_221427829_330000;154000;fixme_Миколаївська_330/LConn1 -- _CN_274597272_330000_CN_221427829_330000/RConn1
  T_221427829_330000;154000;fixme_Миколаївська_330/LConn2 -- _CN_274597272_330000_CN_221427829_330000/RConn2
  _CN_274597272_330000_CN_221427829_330000/RConn3 -- T_221427829_330000;154000;fixme_Миколаївська_330/LConn3 -- bus35/LConn1
  T_184128914_330000;110000;35000;6000_Суми_330/LConn1 -- _CN_184128914_330000_CN_236724724_330000/LConn1
  T_184128914_330000;110000;35000;6000_Суми_330/LConn2 -- _CN_184128914_330000_CN_236724724_330000/LConn2
  _CN_184128914_330000_CN_236724724_330000/LConn3 -- T_184128914_330000;110000;35000;6000_Суми_330/LConn3 -- bus36/LConn1
  _CN_184128914_330000_CN_236724724_330000/RConn1 -- T_236724724_330000;110000;35000_Суми_Північна_330/LConn1 -- _CN_236724724_330000_CN_211101137_330000/RConn1
  _CN_184128914_330000_CN_236724724_330000/RConn2 -- T_236724724_330000;110000;35000_Суми_Північна_330/LConn2 -- _CN_236724724_330000_CN_211101137_330000/RConn2
  _CN_184128914_330000_CN_236724724_330000/RConn3 -- T_236724724_330000;110000;35000_Суми_Північна_330/LConn3 -- _CN_236724724_330000_CN_211101137_330000/RConn3 -- bus37/LConn1
  T_97576344_330000_ПС_“Островская”_330_220_110кВ/LConn1 -- _CN_269527797_330000_CN_97576344_330000/RConn1
  T_97576344_330000_ПС_“Островская”_330_220_110кВ/LConn2 -- _CN_269527797_330000_CN_97576344_330000/RConn2
  _CN_269527797_330000_CN_97576344_330000/RConn3 -- T_97576344_330000_ПС_“Островская”_330_220_110кВ/LConn3 -- bus38/LConn1
  _CN_269527797_330000_CN_123451079_330000/RConn1 -- T_123451079_330000;150000;35000;10000_Мелітопольська_330/LConn1 -- _CN_123451079_330000_CN_228999814_330000/LConn1 -- _CN_123451079_330000_CN_97343458_330000/LConn1 -- _CN_123451079_330000_CN_100454075_330000/LConn1
  _CN_269527797_330000_CN_123451079_330000/RConn2 -- T_123451079_330000;150000;35000;10000_Мелітопольська_330/LConn2 -- _CN_123451079_330000_CN_228999814_330000/LConn2 -- _CN_123451079_330000_CN_97343458_330000/LConn2 -- _CN_123451079_330000_CN_100454075_330000/LConn2
  _CN_269527797_330000_CN_123451079_330000/RConn3 -- T_123451079_330000;150000;35000;10000_Мелітопольська_330/LConn3 -- _CN_123451079_330000_CN_228999814_330000/LConn3 -- _CN_123451079_330000_CN_97343458_330000/LConn3 -- _CN_123451079_330000_CN_100454075_330000/LConn3 -- bus39/LConn1
  _CN_168587285_330000_CN_116452049_330000/RConn1 -- T_116452049_330000;110000_Північна_330/LConn1 -- _CN_116452049_330000_CN_159727866_330000/LConn1
  _CN_168587285_330000_CN_116452049_330000/RConn2 -- T_116452049_330000;110000_Північна_330/LConn2 -- _CN_116452049_330000_CN_159727866_330000/LConn2
  _CN_168587285_330000_CN_116452049_330000/RConn3 -- T_116452049_330000;110000_Північна_330/LConn3 -- _CN_116452049_330000_CN_159727866_330000/LConn3 -- bus40/LConn1
  T_268872470__Славутич_330/LConn1 -- _CN_268872470_330000_CN_295414241_330000/LConn1
  T_268872470__Славутич_330/LConn2 -- _CN_268872470_330000_CN_295414241_330000/LConn2
  _CN_268872470_330000_CN_295414241_330000/LConn3 -- T_268872470__Славутич_330/LConn3 -- bus41/LConn1
  T_295414241__/LConn1 -- _CN_268872470_330000_CN_295414241_330000/RConn1
  T_295414241__/LConn2 -- _CN_268872470_330000_CN_295414241_330000/RConn2
  _CN_268872470_330000_CN_295414241_330000/RConn3 -- T_295414241__/LConn3 -- bus42/LConn1
  _CN_296751070_330000_CN281269420/LConn1 -- T_296751070_330000;110000;10000_Іванівка_330/LConn1 -- _CN_296751070_330000_CN_165762303_330000/RConn1 -- _CN_296751070_330000_CN_176443878_330000/RConn1 -- _CN_296751070_330000_CN_259021748_330000/RConn1
  _CN_296751070_330000_CN281269420/LConn2 -- T_296751070_330000;110000;10000_Іванівка_330/LConn2 -- _CN_296751070_330000_CN_165762303_330000/RConn2 -- _CN_296751070_330000_CN_176443878_330000/RConn2 -- _CN_296751070_330000_CN_259021748_330000/RConn2
  _CN_296751070_330000_CN281269420/LConn3 -- T_296751070_330000;110000;10000_Іванівка_330/LConn3 -- _CN_296751070_330000_CN_165762303_330000/RConn3 -- _CN_296751070_330000_CN_176443878_330000/RConn3 -- _CN_296751070_330000_CN_259021748_330000/RConn3 -- bus43/LConn1
  _CN_296751070_330000_CN281269420/RConn1 -- G_281269420_Кураховська_ТЭС/RConn1 -- _CN_209879378_330000_CN281269420/RConn1
  _CN_296751070_330000_CN281269420/RConn2 -- G_281269420_Кураховська_ТЭС/RConn2 -- _CN_209879378_330000_CN281269420/RConn2
  _CN_296751070_330000_CN281269420/RConn3 -- G_281269420_Кураховська_ТЭС/RConn3 -- _CN_209879378_330000_CN281269420/RConn3 -- bus44/LConn1
  T_295492532_330000;110000;10000_Лісова_330/LConn1 -- _CN_295492532_330000_CN_209425313_330000/LConn1
  T_295492532_330000;110000;10000_Лісова_330/LConn2 -- _CN_295492532_330000_CN_209425313_330000/LConn2
  _CN_295492532_330000_CN_209425313_330000/LConn3 -- T_295492532_330000;110000;10000_Лісова_330/LConn3 -- bus45/LConn1
  _CN_295492532_330000_CN_209425313_330000/RConn1 -- T_209425313_330000;150000;35000;10000_Житомирська_330/LConn1 -- _CN_209425313_330000_CN_295492533_330000/LConn1
  _CN_295492532_330000_CN_209425313_330000/RConn2 -- T_209425313_330000;150000;35000;10000_Житомирська_330/LConn2 -- _CN_209425313_330000_CN_295492533_330000/LConn2
  _CN_295492532_330000_CN_209425313_330000/RConn3 -- T_209425313_330000;150000;35000;10000_Житомирська_330/LConn3 -- _CN_209425313_330000_CN_295492533_330000/LConn3 -- bus46/LConn1
  _CN_274598688_330000_CN_28878309_330000/RConn1 -- T_28878309__/LConn1 -- _CN_107808612_330000_CN_28878309_330000/LConn1 -- _CN_28878309_330000_CN_296062375_330000/LConn1 -- _CN_28878309_330000_CN_202269421_330000/LConn1 -- _CN_28878309_330000_CN136057743/LConn1 -- _CN_325748197_330000_CN_28878309_330000/LConn1 -- _CN_296062370_330000_CN_28878309_330000/LConn1
  _CN_274598688_330000_CN_28878309_330000/RConn2 -- T_28878309__/LConn2 -- _CN_107808612_330000_CN_28878309_330000/LConn2 -- _CN_28878309_330000_CN_296062375_330000/LConn2 -- _CN_28878309_330000_CN_202269421_330000/LConn2 -- _CN_28878309_330000_CN136057743/LConn2 -- _CN_325748197_330000_CN_28878309_330000/LConn2 -- _CN_296062370_330000_CN_28878309_330000/LConn2
  _CN_274598688_330000_CN_28878309_330000/RConn3 -- T_28878309__/LConn3 -- _CN_107808612_330000_CN_28878309_330000/LConn3 -- _CN_28878309_330000_CN_296062375_330000/LConn3 -- _CN_28878309_330000_CN_202269421_330000/LConn3 -- _CN_28878309_330000_CN136057743/LConn3 -- bus47/LConn1 -- _CN_325748197_330000_CN_28878309_330000/LConn3 -- _CN_296062370_330000_CN_28878309_330000/LConn3
  T_296496011_330000;220000;150000;35000_Трихати_330/LConn1 -- _CN_274598688_330000_CN_296496011_330000/RConn1
  T_296496011_330000;220000;150000;35000_Трихати_330/LConn2 -- _CN_274598688_330000_CN_296496011_330000/RConn2
  _CN_274598688_330000_CN_296496011_330000/RConn3 -- T_296496011_330000;220000;150000;35000_Трихати_330/LConn3 -- bus48/LConn1
  T_295492533__Шепетівка_330/LConn1 -- _CN_209425313_330000_CN_295492533_330000/RConn1
  T_295492533__Шепетівка_330/LConn2 -- _CN_209425313_330000_CN_295492533_330000/RConn2
  _CN_209425313_330000_CN_295492533_330000/RConn3 -- T_295492533__Шепетівка_330/LConn3 -- bus49/LConn1
  "T_207700515_330000_ПС_330_кВ_\"Зміївська_ТЕС\""/LConn1 -- _CN_207700515_330000_CN164920951/LConn1
  "T_207700515_330000_ПС_330_кВ_\"Зміївська_ТЕС\""/LConn2 -- _CN_207700515_330000_CN164920951/LConn2
  _CN_207700515_330000_CN164920951/LConn3 -- "T_207700515_330000_ПС_330_кВ_\"Зміївська_ТЕС\""/LConn3 -- bus50/LConn1
  _CN_207700515_330000_CN164920951/RConn1 -- G_164920951_Слов'янська_ТЕЦ/RConn1 -- _CN_130513926_330000_CN164920951/LConn1
  _CN_207700515_330000_CN164920951/RConn2 -- G_164920951_Слов'янська_ТЕЦ/RConn2 -- _CN_130513926_330000_CN164920951/LConn2
  _CN_207700515_330000_CN164920951/RConn3 -- G_164920951_Слов'янська_ТЕЦ/RConn3 -- _CN_130513926_330000_CN164920951/LConn3 -- bus51/LConn1
  _CN_130513926_330000_CN_188001625_330000/RConn1 -- T_130513926_330000;110000;10000_«Травнева»_330_110_кВ/LConn1 -- _CN_130513926_330000_CN164920951/RConn1 -- _CN_130513926_330000_CN_219508915_330000/RConn1
  _CN_130513926_330000_CN_188001625_330000/RConn2 -- T_130513926_330000;110000;10000_«Травнева»_330_110_кВ/LConn2 -- _CN_130513926_330000_CN164920951/RConn2 -- _CN_130513926_330000_CN_219508915_330000/RConn2
  _CN_130513926_330000_CN_188001625_330000/RConn3 -- T_130513926_330000;110000;10000_«Травнева»_330_110_кВ/LConn3 -- _CN_130513926_330000_CN164920951/RConn3 -- _CN_130513926_330000_CN_219508915_330000/RConn3 -- bus52/LConn1
  "T_158848422_330000;110000;10000_ПС_330_кВ_\"Поляна\""/LConn1 -- _CN_158848422_330000_CN73199860/LConn1
  "T_158848422_330000;110000;10000_ПС_330_кВ_\"Поляна\""/LConn2 -- _CN_158848422_330000_CN73199860/LConn2
  _CN_158848422_330000_CN73199860/LConn3 -- "T_158848422_330000;110000;10000_ПС_330_кВ_\"Поляна\""/LConn3 -- bus53/LConn1
  G_73199860_Канівська_ГЕС/RConn1 -- _CN_158848422_330000_CN73199860/RConn1
  G_73199860_Канівська_ГЕС/RConn2 -- _CN_158848422_330000_CN73199860/RConn2
  _CN_158848422_330000_CN73199860/RConn3 -- G_73199860_Канівська_ГЕС/RConn3 -- bus54/LConn1
  _CN_171816615_330000_CN_290562726_330000/LConn1 -- T_171816615_330000;110000;35000;10000_Червоноармійська_330/LConn1 -- _CN_171816615_330000_CN_188001625_330000/RConn1
  _CN_171816615_330000_CN_290562726_330000/LConn2 -- T_171816615_330000;110000;35000;10000_Червоноармійська_330/LConn2 -- _CN_171816615_330000_CN_188001625_330000/RConn2
  _CN_171816615_330000_CN_290562726_330000/LConn3 -- T_171816615_330000;110000;35000;10000_Червоноармійська_330/LConn3 -- _CN_171816615_330000_CN_188001625_330000/RConn3 -- bus55/LConn1
  T_290562726_330000;150000;35000;6000_Павлоградська_330/LConn1 -- _CN_171816615_330000_CN_290562726_330000/RConn1
  T_290562726_330000;150000;35000;6000_Павлоградська_330/LConn2 -- _CN_171816615_330000_CN_290562726_330000/RConn2
  _CN_171816615_330000_CN_290562726_330000/RConn3 -- T_290562726_330000;150000;35000;6000_Павлоградська_330/LConn3 -- bus56/LConn1
  _CN_259242024_330000_CN_179967275_330000/LConn1 -- T_259242024__ОРУ_330_154_кВ/LConn1 -- _CN_259242024_330000_CN259242291/LConn1
  _CN_259242024_330000_CN_179967275_330000/LConn2 -- T_259242024__ОРУ_330_154_кВ/LConn2 -- _CN_259242024_330000_CN259242291/LConn2
  _CN_259242024_330000_CN_179967275_330000/LConn3 -- T_259242024__ОРУ_330_154_кВ/LConn3 -- _CN_259242024_330000_CN259242291/LConn3 -- bus57/LConn1
  _CN_259242024_330000_CN_179967275_330000/RConn1 -- T_179967275_330000;150000;10000;6000_Першотравнева_330/LConn1 -- _CN_179967275_330000_CN_251145082_330000/LConn1 -- _CN_179967275_330000_CN_148566248_330000/LConn1
  _CN_259242024_330000_CN_179967275_330000/RConn2 -- T_179967275_330000;150000;10000;6000_Першотравнева_330/LConn2 -- _CN_179967275_330000_CN_251145082_330000/LConn2 -- _CN_179967275_330000_CN_148566248_330000/LConn2
  _CN_259242024_330000_CN_179967275_330000/RConn3 -- T_179967275_330000;150000;10000;6000_Першотравнева_330/LConn3 -- _CN_179967275_330000_CN_251145082_330000/LConn3 -- _CN_179967275_330000_CN_148566248_330000/LConn3 -- bus58/LConn1
  G_259242291_Кременчуцька_ГЕС/RConn1 -- _CN_259242024_330000_CN259242291/RConn1
  G_259242291_Кременчуцька_ГЕС/RConn2 -- _CN_259242024_330000_CN259242291/RConn2
  _CN_259242024_330000_CN259242291/RConn3 -- G_259242291_Кременчуцька_ГЕС/RConn3 -- bus59/LConn1
  _CN_179967275_330000_CN_251145082_330000/RConn1 -- T_251145082_330000;150000;35000_Рудна_330/LConn1 -- _CN_296062370_330000_CN_251145082_330000/LConn1
  _CN_179967275_330000_CN_251145082_330000/RConn2 -- T_251145082_330000;150000;35000_Рудна_330/LConn2 -- _CN_296062370_330000_CN_251145082_330000/LConn2
  _CN_179967275_330000_CN_251145082_330000/RConn3 -- T_251145082_330000;150000;35000_Рудна_330/LConn3 -- _CN_296062370_330000_CN_251145082_330000/LConn3 -- bus60/LConn1
  T_148566248_330000;150000;10000_Південна_330/LConn1 -- _CN_179967275_330000_CN_148566248_330000/RConn1
  T_148566248_330000;150000;10000_Південна_330/LConn2 -- _CN_179967275_330000_CN_148566248_330000/RConn2
  _CN_179967275_330000_CN_148566248_330000/RConn3 -- T_148566248_330000;150000;10000_Південна_330/LConn3 -- bus61/LConn1
  _CN_172507826_330000_CN_289148613_330000/LConn1 -- T_172507826_750000;330000;15000_Південнодонбаська_750/LConn1 -- _CN_172507826_330000_CN_259021748_330000/RConn1
  _CN_172507826_330000_CN_289148613_330000/LConn2 -- T_172507826_750000;330000;15000_Південнодонбаська_750/LConn2 -- _CN_172507826_330000_CN_259021748_330000/RConn2
  _CN_172507826_330000_CN_289148613_330000/LConn3 -- T_172507826_750000;330000;15000_Південнодонбаська_750/LConn3 -- _CN_172507826_330000_CN_259021748_330000/RConn3 -- bus62/LConn1
  _CN_172507826_330000_CN_289148613_330000/RConn1 -- T_289148613_330000;110000;10000_Мирна_330/LConn1 -- _CN_289148613_330000_CN_259021748_330000/RConn1
  _CN_172507826_330000_CN_289148613_330000/RConn2 -- T_289148613_330000;110000;10000_Мирна_330/LConn2 -- _CN_289148613_330000_CN_259021748_330000/RConn2
  _CN_172507826_330000_CN_289148613_330000/RConn3 -- T_289148613_330000;110000;10000_Мирна_330/LConn3 -- _CN_289148613_330000_CN_259021748_330000/RConn3 -- bus63/LConn1
  _CN_237532980_330000_CN_159727866_330000/RConn1 -- T_159727866_330000;110000_пс_330_110_КВ_«Новокиевская»/LConn1 -- _CN_152182710_330000_CN_159727866_330000/LConn1 -- _CN_116452049_330000_CN_159727866_330000/RConn1
  _CN_237532980_330000_CN_159727866_330000/RConn2 -- T_159727866_330000;110000_пс_330_110_КВ_«Новокиевская»/LConn2 -- _CN_152182710_330000_CN_159727866_330000/LConn2 -- _CN_116452049_330000_CN_159727866_330000/RConn2
  _CN_237532980_330000_CN_159727866_330000/RConn3 -- T_159727866_330000;110000_пс_330_110_КВ_«Новокиевская»/LConn3 -- _CN_152182710_330000_CN_159727866_330000/LConn3 -- _CN_116452049_330000_CN_159727866_330000/RConn3 -- bus64/LConn1
  T_152182710_330000;110000;35000;fixme_Жовтнева_330/LConn1 -- _CN_152182710_330000_CN_159727866_330000/RConn1
  T_152182710_330000;110000;35000;fixme_Жовтнева_330/LConn2 -- _CN_152182710_330000_CN_159727866_330000/RConn2
  _CN_152182710_330000_CN_159727866_330000/RConn3 -- T_152182710_330000;110000;35000;fixme_Жовтнева_330/LConn3 -- bus65/LConn1
  T_150153410_330000;150000;35000;6000_Прометей_330/LConn1 -- _CN_150153410_330000_CN_165767625_330000/LConn1
  T_150153410_330000;150000;35000;6000_Прометей_330/LConn2 -- _CN_150153410_330000_CN_165767625_330000/LConn2
  _CN_150153410_330000_CN_165767625_330000/LConn3 -- T_150153410_330000;150000;35000;6000_Прометей_330/LConn3 -- bus66/LConn1
  T_165767625_750000;330000;15000_Дніпровська_750/LConn1 -- _CN_150153410_330000_CN_165767625_330000/RConn1
  T_165767625_750000;330000;15000_Дніпровська_750/LConn2 -- _CN_150153410_330000_CN_165767625_330000/RConn2
  _CN_150153410_330000_CN_165767625_330000/RConn3 -- T_165767625_750000;330000;15000_Дніпровська_750/LConn3 -- bus67/LConn1
  T_228999814_330000;150000;35000_Молочанська_330/LConn1 -- _CN_123451079_330000_CN_228999814_330000/RConn1
  T_228999814_330000;150000;35000_Молочанська_330/LConn2 -- _CN_123451079_330000_CN_228999814_330000/RConn2
  _CN_123451079_330000_CN_228999814_330000/RConn3 -- T_228999814_330000;150000;35000_Молочанська_330/LConn3 -- bus68/LConn1
  T_97343458_330000;220000;110000_Джанкой_330/LConn1 -- _CN_123451079_330000_CN_97343458_330000/RConn1
  T_97343458_330000;220000;110000_Джанкой_330/LConn2 -- _CN_123451079_330000_CN_97343458_330000/RConn2
  _CN_123451079_330000_CN_97343458_330000/RConn3 -- T_97343458_330000;220000;110000_Джанкой_330/LConn3 -- bus69/LConn1
  T_100454075__/LConn1 -- _CN_123451079_330000_CN_100454075_330000/RConn1
  T_100454075__/LConn2 -- _CN_123451079_330000_CN_100454075_330000/RConn2
  _CN_123451079_330000_CN_100454075_330000/RConn3 -- T_100454075__/LConn3 -- bus70/LConn1
  _CN_296062370_330000_CN_251145082_330000/RConn1 -- T_296062370_330000;150000;35000_Кварцит_330/LConn1 -- _CN_296062370_330000_CN_28878309_330000/RConn1 -- _CN_296062370_330000_CN_202269421_330000/LConn1
  _CN_296062370_330000_CN_251145082_330000/RConn2 -- T_296062370_330000;150000;35000_Кварцит_330/LConn2 -- _CN_296062370_330000_CN_28878309_330000/RConn2 -- _CN_296062370_330000_CN_202269421_330000/LConn2
  _CN_296062370_330000_CN_251145082_330000/RConn3 -- T_296062370_330000;150000;35000_Кварцит_330/LConn3 -- _CN_296062370_330000_CN_28878309_330000/RConn3 -- bus71/LConn1 -- _CN_296062370_330000_CN_202269421_330000/LConn3
  _CN_296062370_330000_CN_202269421_330000/RConn1 -- T_202269421_330000;150000;10000_Українка_330/LConn1 -- _CN_28878309_330000_CN_202269421_330000/RConn1
  _CN_296062370_330000_CN_202269421_330000/RConn2 -- T_202269421_330000;150000;10000_Українка_330/LConn2 -- _CN_28878309_330000_CN_202269421_330000/RConn2
  _CN_296062370_330000_CN_202269421_330000/RConn3 -- T_202269421_330000;150000;10000_Українка_330/LConn3 -- _CN_28878309_330000_CN_202269421_330000/RConn3 -- bus72/LConn1
  T_325748197__/LConn1 -- _CN_325748197_330000_CN_28878309_330000/RConn1
  T_325748197__/LConn2 -- _CN_325748197_330000_CN_28878309_330000/RConn2
  _CN_325748197_330000_CN_28878309_330000/RConn3 -- T_325748197__/LConn3 -- bus73/LConn1
  T_107808612__/LConn1 -- _CN_107808612_330000_CN_28878309_330000/RConn1
  T_107808612__/LConn2 -- _CN_107808612_330000_CN_28878309_330000/RConn2
  _CN_107808612_330000_CN_28878309_330000/RConn3 -- T_107808612__/LConn3 -- bus74/LConn1
  T_296062375_330000;150000;35000_Побузька_330/LConn1 -- _CN_28878309_330000_CN_296062375_330000/RConn1
  T_296062375_330000;150000;35000_Побузька_330/LConn2 -- _CN_28878309_330000_CN_296062375_330000/RConn2
  _CN_28878309_330000_CN_296062375_330000/RConn3 -- T_296062375_330000;150000;35000_Побузька_330/LConn3 -- bus75/LConn1
  G_136057743_Ташлицька_ГАЕС/RConn1 -- _CN_28878309_330000_CN136057743/RConn1
  G_136057743_Ташлицька_ГАЕС/RConn2 -- _CN_28878309_330000_CN136057743/RConn2
  _CN_28878309_330000_CN136057743/RConn3 -- G_136057743_Ташлицька_ГАЕС/RConn3 -- bus76/LConn1
  T_107811059_750000;330000_/LConn1 -- _CN_107811059_330000_CN28878854/LConn1
  T_107811059_750000;330000_/LConn2 -- _CN_107811059_330000_CN28878854/LConn2
  _CN_107811059_330000_CN28878854/LConn3 -- T_107811059_750000;330000_/LConn3 -- bus77/LConn1
  G_28878854_Рівненська_АЕС/RConn1 -- _CN_107811059_330000_CN28878854/RConn1
  G_28878854_Рівненська_АЕС/RConn2 -- _CN_107811059_330000_CN28878854/RConn2
  _CN_107811059_330000_CN28878854/RConn3 -- G_28878854_Рівненська_АЕС/RConn3 -- bus78/LConn1
  T_182915221_330000;110000;10000_Харцизька_330/RConn1 -- L_182915221/LConn1
  T_182915221_330000;110000;10000_Харцизька_330/RConn2 -- L_182915221/LConn2
  L_182915221/LConn3 -- T_182915221_330000;110000;10000_Харцизька_330/RConn3 -- bus79/LConn1
  T_259021748_330000;110000;10000_Зоря_330/RConn1 -- L_259021748/LConn1
  T_259021748_330000;110000;10000_Зоря_330/RConn2 -- L_259021748/LConn2
  L_259021748/LConn3 -- T_259021748_330000;110000;10000_Зоря_330/RConn3 -- bus80/LConn1
  T_165762303_330000;220000;110000;35000;6000_Чайкіне_330/RConn1 -- L_165762303/LConn1
  T_165762303_330000;220000;110000;35000;6000_Чайкіне_330/RConn2 -- L_165762303/LConn2
  L_165762303/LConn3 -- T_165762303_330000;220000;110000;35000;6000_Чайкіне_330/RConn3 -- bus81/LConn1
  T_155861889__/RConn1 -- L_155861889/LConn1
  T_155861889__/RConn2 -- L_155861889/LConn2
  L_155861889/LConn3 -- T_155861889__/RConn3 -- bus82/LConn1
  T_155861891__/RConn1 -- L_155861891/LConn1
  T_155861891__/RConn2 -- L_155861891/LConn2
  L_155861891/LConn3 -- T_155861891__/RConn3 -- bus83/LConn1
  T_274598688__Аджалик_330/RConn1 -- L_274598688/LConn1
  T_274598688__Аджалик_330/RConn2 -- L_274598688/LConn2
  L_274598688/LConn3 -- T_274598688__Аджалик_330/RConn3 -- bus84/LConn1
  T_292523027__/RConn1 -- L_292523027/LConn1
  T_292523027__/RConn2 -- L_292523027/LConn2
  L_292523027/LConn3 -- T_292523027__/RConn3 -- bus85/LConn1
  T_135644235_400000;330000;220000;110000;35000_Михайлівка_330/RConn1 -- L_135644235/LConn1
  T_135644235_400000;330000;220000;110000;35000_Михайлівка_330/RConn2 -- L_135644235/LConn2
  L_135644235/LConn3 -- T_135644235_400000;330000;220000;110000;35000_Михайлівка_330/RConn3 -- bus86/LConn1
  T_219508915_750000;500000;330000;15000_Донбаська_750/RConn1 -- L_219508915/LConn1
  T_219508915_750000;500000;330000;15000_Донбаська_750/RConn2 -- L_219508915/LConn2
  L_219508915/LConn3 -- T_219508915_750000;500000;330000;15000_Донбаська_750/RConn3 -- bus87/LConn1
  T_188001625_330000;110000;35000;10000_«Центральна»_330_110_35_кВ/RConn1 -- L_188001625/LConn1
  T_188001625_330000;110000;35000;10000_«Центральна»_330_110_35_кВ/RConn2 -- L_188001625/LConn2
  L_188001625/LConn3 -- T_188001625_330000;110000;35000;10000_«Центральна»_330_110_35_кВ/RConn3 -- bus88/LConn1
  T_176443878_330000;110000;35000;10000_Макіївська/RConn1 -- L_176443878/LConn1
  T_176443878_330000;110000;35000;10000_Макіївська/RConn2 -- L_176443878/LConn2
  L_176443878/LConn3 -- T_176443878_330000;110000;35000;10000_Макіївська/RConn3 -- bus89/LConn1
  "T_99234566_330000;110000_ПС_330_110_кВ_\"Білоцерківська\""/RConn1 -- L_99234566/LConn1
  "T_99234566_330000;110000_ПС_330_110_кВ_\"Білоцерківська\""/RConn2 -- L_99234566/LConn2
  L_99234566/LConn3 -- "T_99234566_330000;110000_ПС_330_110_кВ_\"Білоцерківська\""/RConn3 -- bus90/LConn1
  T_211109125_330000;110000;35000_Козятин_330/RConn1 -- L_211109125/LConn1
  T_211109125_330000;110000;35000_Козятин_330/RConn2 -- L_211109125/LConn2
  L_211109125/LConn3 -- T_211109125_330000;110000;35000_Козятин_330/RConn3 -- bus91/LConn1
  T_157927169_330000;150000;10000_ПС_Дніпропетровська_330/RConn1 -- L_157927169/LConn1
  T_157927169_330000;150000;10000_ПС_Дніпропетровська_330/RConn2 -- L_157927169/LConn2
  L_157927169/LConn3 -- T_157927169_330000;150000;10000_ПС_Дніпропетровська_330/RConn3 -- bus92/LConn1
  T_209879378_750000;330000;35000;15000_Запорізька_750/RConn1 -- L_209879378/LConn1
  T_209879378_750000;330000;35000;15000_Запорізька_750/RConn2 -- L_209879378/LConn2
  L_209879378/LConn3 -- T_209879378_750000;330000;35000;15000_Запорізька_750/RConn3 -- bus93/LConn1
  T_292523016__Лозова/RConn1 -- L_292523016/LConn1
  T_292523016__Лозова/RConn2 -- L_292523016/LConn2
  L_292523016/LConn3 -- T_292523016__Лозова/RConn3 -- bus94/LConn1
  T_203926610_330000;110000;10000_Первомайськ_330/RConn1 -- L_203926610/LConn1
  T_203926610_330000;110000;10000_Первомайськ_330/RConn2 -- L_203926610/LConn2
  L_203926610/LConn3 -- T_203926610_330000;110000;10000_Первомайськ_330/RConn3 -- bus95/LConn1
  T_104864777__/RConn1 -- L_104864777/LConn1
  T_104864777__/RConn2 -- L_104864777/LConn2
  L_104864777/LConn3 -- T_104864777__/RConn3 -- bus96/LConn1
  T_237532980__/RConn1 -- L_237532980/LConn1
  T_237532980__/RConn2 -- L_237532980/LConn2
  L_237532980/LConn3 -- T_237532980__/RConn3 -- bus97/LConn1
  T_168587285__/RConn1 -- L_168587285/LConn1
  T_168587285__/RConn2 -- L_168587285/LConn2
  L_168587285/LConn3 -- T_168587285__/RConn3 -- bus98/LConn1
  T_74481802__Вінниця_330/RConn1 -- L_74481802/LConn1
  T_74481802__Вінниця_330/RConn2 -- L_74481802/LConn2
  L_74481802/LConn3 -- T_74481802__Вінниця_330/RConn3 -- bus99/LConn1
  T_70994591_750000;330000;110000_Вінниця_750/RConn1 -- L_70994591/LConn1
  T_70994591_750000;330000;110000_Вінниця_750/RConn2 -- L_70994591/LConn2
  L_70994591/LConn3 -- T_70994591_750000;330000;110000_Вінниця_750/RConn3 -- bus100/LConn1
  T_212379146__Бар_330/RConn1 -- L_212379146/LConn1
  T_212379146__Бар_330/RConn2 -- L_212379146/LConn2
  L_212379146/LConn3 -- T_212379146__Бар_330/RConn3 -- bus101/LConn1
  "T_169821963_330000_ПС_330_кВ_\"Чернівці\""/RConn1 -- L_169821963/LConn1
  "T_169821963_330000_ПС_330_кВ_\"Чернівці\""/RConn2 -- L_169821963/LConn2
  L_169821963/LConn3 -- "T_169821963_330000_ПС_330_кВ_\"Чернівці\""/RConn3 -- bus102/LConn1
  T_275503522__Кам’янець_Подільська_330/RConn1 -- L_275503522/LConn1
  T_275503522__Кам’янець_Подільська_330/RConn2 -- L_275503522/LConn2
  L_275503522/LConn3 -- T_275503522__Кам’янець_Подільська_330/RConn3 -- bus103/LConn1
  "T_215079308_330000_Підстанція_\"Полтава\""/RConn1 -- L_215079308/LConn1
  "T_215079308_330000_Підстанція_\"Полтава\""/RConn2 -- L_215079308/LConn2
  L_215079308/LConn3 -- "T_215079308_330000_Підстанція_\"Полтава\""/RConn3 -- bus104/LConn1
  "T_269056567_330000_ПС_330_154_35_10_кВ_\"Кременчук\""/RConn1 -- L_269056567/LConn1
  "T_269056567_330000_ПС_330_154_35_10_кВ_\"Кременчук\""/RConn2 -- L_269056567/LConn2
  L_269056567/LConn3 -- "T_269056567_330000_ПС_330_154_35_10_кВ_\"Кременчук\""/RConn3 -- bus105/LConn1
  T_294742933__Миргород_330/RConn1 -- L_294742933/LConn1
  T_294742933__Миргород_330/RConn2 -- L_294742933/LConn2
  L_294742933/LConn3 -- T_294742933__Миргород_330/RConn3 -- bus106/LConn1
  T_211101137__Північноукраїнська_750/RConn1 -- L_211101137/LConn1
  T_211101137__Північноукраїнська_750/RConn2 -- L_211101137/LConn2
  L_211101137/LConn3 -- T_211101137__Північноукраїнська_750/RConn3 -- bus107/LConn1
  T_274597272_330000;150000;35000_Херсонська_330/RConn1 -- L_274597272/LConn1
  T_274597272_330000;150000;35000_Херсонська_330/RConn2 -- L_274597272/LConn2
  L_274597272/LConn3 -- T_274597272_330000;150000;35000_Херсонська_330/RConn3 -- bus108/LConn1
  "T_269527797_330000;220000;154000;35000;6000_ПС_330_220_150_кВ_\"Новокаховська\""/RConn1 -- L_269527797/LConn1
  "T_269527797_330000;220000;154000;35000;6000_ПС_330_220_150_кВ_\"Новокаховська\""/RConn2 -- L_269527797/LConn2
  L_269527797/LConn3 -- "T_269527797_330000;220000;154000;35000;6000_ПС_330_220_150_кВ_\"Новокаховська\""/RConn3 -- bus109/LConn1
  T_221427829_330000;154000;fixme_Миколаївська_330/RConn1 -- L_221427829/LConn1
  T_221427829_330000;154000;fixme_Миколаївська_330/RConn2 -- L_221427829/LConn2
  L_221427829/LConn3 -- T_221427829_330000;154000;fixme_Миколаївська_330/RConn3 -- bus110/LConn1
  T_184128914_330000;110000;35000;6000_Суми_330/RConn1 -- L_184128914/LConn1
  T_184128914_330000;110000;35000;6000_Суми_330/RConn2 -- L_184128914/LConn2
  L_184128914/LConn3 -- T_184128914_330000;110000;35000;6000_Суми_330/RConn3 -- bus111/LConn1
  T_236724724_330000;110000;35000_Суми_Північна_330/RConn1 -- L_236724724/LConn1
  T_236724724_330000;110000;35000_Суми_Північна_330/RConn2 -- L_236724724/LConn2
  L_236724724/LConn3 -- T_236724724_330000;110000;35000_Суми_Північна_330/RConn3 -- bus112/LConn1
  T_97576344_330000_ПС_“Островская”_330_220_110кВ/RConn1 -- L_97576344/LConn1
  T_97576344_330000_ПС_“Островская”_330_220_110кВ/RConn2 -- L_97576344/LConn2
  L_97576344/LConn3 -- T_97576344_330000_ПС_“Островская”_330_220_110кВ/RConn3 -- bus113/LConn1
  T_123451079_330000;150000;35000;10000_Мелітопольська_330/RConn1 -- L_123451079/LConn1
  T_123451079_330000;150000;35000;10000_Мелітопольська_330/RConn2 -- L_123451079/LConn2
  L_123451079/LConn3 -- T_123451079_330000;150000;35000;10000_Мелітопольська_330/RConn3 -- bus114/LConn1
  T_116452049_330000;110000_Північна_330/RConn1 -- L_116452049/LConn1
  T_116452049_330000;110000_Північна_330/RConn2 -- L_116452049/LConn2
  L_116452049/LConn3 -- T_116452049_330000;110000_Північна_330/RConn3 -- bus115/LConn1
  T_268872470__Славутич_330/RConn1 -- L_268872470/LConn1
  T_268872470__Славутич_330/RConn2 -- L_268872470/LConn2
  L_268872470/LConn3 -- T_268872470__Славутич_330/RConn3 -- bus116/LConn1
  T_295414241__/RConn1 -- L_295414241/LConn1
  T_295414241__/RConn2 -- L_295414241/LConn2
  L_295414241/LConn3 -- T_295414241__/RConn3 -- bus117/LConn1
  T_296751070_330000;110000;10000_Іванівка_330/RConn1 -- L_296751070/LConn1
  T_296751070_330000;110000;10000_Іванівка_330/RConn2 -- L_296751070/LConn2
  L_296751070/LConn3 -- T_296751070_330000;110000;10000_Іванівка_330/RConn3 -- bus118/LConn1
  T_295492532_330000;110000;10000_Лісова_330/RConn1 -- L_295492532/LConn1
  T_295492532_330000;110000;10000_Лісова_330/RConn2 -- L_295492532/LConn2
  L_295492532/LConn3 -- T_295492532_330000;110000;10000_Лісова_330/RConn3 -- bus119/LConn1
  T_209425313_330000;150000;35000;10000_Житомирська_330/RConn1 -- L_209425313/LConn1
  T_209425313_330000;150000;35000;10000_Житомирська_330/RConn2 -- L_209425313/LConn2
  L_209425313/LConn3 -- T_209425313_330000;150000;35000;10000_Житомирська_330/RConn3 -- bus120/LConn1
  T_28878309__/RConn1 -- L_28878309/LConn1
  T_28878309__/RConn2 -- L_28878309/LConn2
  L_28878309/LConn3 -- T_28878309__/RConn3 -- bus121/LConn1
  T_296496011_330000;220000;150000;35000_Трихати_330/RConn1 -- L_296496011/LConn1
  T_296496011_330000;220000;150000;35000_Трихати_330/RConn2 -- L_296496011/LConn2
  L_296496011/LConn3 -- T_296496011_330000;220000;150000;35000_Трихати_330/RConn3 -- bus122/LConn1
  T_295492533__Шепетівка_330/RConn1 -- L_295492533/LConn1
  T_295492533__Шепетівка_330/RConn2 -- L_295492533/LConn2
  L_295492533/LConn3 -- T_295492533__Шепетівка_330/RConn3 -- bus123/LConn1
  "T_207700515_330000_ПС_330_кВ_\"Зміївська_ТЕС\""/RConn1 -- L_207700515/LConn1
  "T_207700515_330000_ПС_330_кВ_\"Зміївська_ТЕС\""/RConn2 -- L_207700515/LConn2
  L_207700515/LConn3 -- "T_207700515_330000_ПС_330_кВ_\"Зміївська_ТЕС\""/RConn3 -- bus124/LConn1
  T_130513926_330000;110000;10000_«Травнева»_330_110_кВ/RConn1 -- L_130513926/LConn1
  T_130513926_330000;110000;10000_«Травнева»_330_110_кВ/RConn2 -- L_130513926/LConn2
  L_130513926/LConn3 -- T_130513926_330000;110000;10000_«Травнева»_330_110_кВ/RConn3 -- bus125/LConn1
  "T_158848422_330000;110000;10000_ПС_330_кВ_\"Поляна\""/RConn1 -- L_158848422/LConn1
  "T_158848422_330000;110000;10000_ПС_330_кВ_\"Поляна\""/RConn2 -- L_158848422/LConn2
  L_158848422/LConn3 -- "T_158848422_330000;110000;10000_ПС_330_кВ_\"Поляна\""/RConn3 -- bus126/LConn1
  T_171816615_330000;110000;35000;10000_Червоноармійська_330/RConn1 -- L_171816615/LConn1
  T_171816615_330000;110000;35000;10000_Червоноармійська_330/RConn2 -- L_171816615/LConn2
  L_171816615/LConn3 -- T_171816615_330000;110000;35000;10000_Червоноармійська_330/RConn3 -- bus127/LConn1
  T_290562726_330000;150000;35000;6000_Павлоградська_330/RConn1 -- L_290562726/LConn1
  T_290562726_330000;150000;35000;6000_Павлоградська_330/RConn2 -- L_290562726/LConn2
  L_290562726/LConn3 -- T_290562726_330000;150000;35000;6000_Павлоградська_330/RConn3 -- bus128/LConn1
  T_259242024__ОРУ_330_154_кВ/RConn1 -- L_259242024/LConn1
  T_259242024__ОРУ_330_154_кВ/RConn2 -- L_259242024/LConn2
  L_259242024/LConn3 -- T_259242024__ОРУ_330_154_кВ/RConn3 -- bus129/LConn1
  T_179967275_330000;150000;10000;6000_Першотравнева_330/RConn1 -- L_179967275/LConn1
  T_179967275_330000;150000;10000;6000_Першотравнева_330/RConn2 -- L_179967275/LConn2
  L_179967275/LConn3 -- T_179967275_330000;150000;10000;6000_Першотравнева_330/RConn3 -- bus130/LConn1
  T_251145082_330000;150000;35000_Рудна_330/RConn1 -- L_251145082/LConn1
  T_251145082_330000;150000;35000_Рудна_330/RConn2 -- L_251145082/LConn2
  L_251145082/LConn3 -- T_251145082_330000;150000;35000_Рудна_330/RConn3 -- bus131/LConn1
  T_148566248_330000;150000;10000_Південна_330/RConn1 -- L_148566248/LConn1
  T_148566248_330000;150000;10000_Південна_330/RConn2 -- L_148566248/LConn2
  L_148566248/LConn3 -- T_148566248_330000;150000;10000_Південна_330/RConn3 -- bus132/LConn1
  T_172507826_750000;330000;15000_Південнодонбаська_750/RConn1 -- L_172507826/LConn1
  T_172507826_750000;330000;15000_Південнодонбаська_750/RConn2 -- L_172507826/LConn2
  L_172507826/LConn3 -- T_172507826_750000;330000;15000_Південнодонбаська_750/RConn3 -- bus133/LConn1
  T_289148613_330000;110000;10000_Мирна_330/RConn1 -- L_289148613/LConn1
  T_289148613_330000;110000;10000_Мирна_330/RConn2 -- L_289148613/LConn2
  L_289148613/LConn3 -- T_289148613_330000;110000;10000_Мирна_330/RConn3 -- bus134/LConn1
  T_159727866_330000;110000_пс_330_110_КВ_«Новокиевская»/RConn1 -- L_159727866/LConn1
  T_159727866_330000;110000_пс_330_110_КВ_«Новокиевская»/RConn2 -- L_159727866/LConn2
  L_159727866/LConn3 -- T_159727866_330000;110000_пс_330_110_КВ_«Новокиевская»/RConn3 -- bus135/LConn1
  T_152182710_330000;110000;35000;fixme_Жовтнева_330/RConn1 -- L_152182710/LConn1
  T_152182710_330000;110000;35000;fixme_Жовтнева_330/RConn2 -- L_152182710/LConn2
  L_152182710/LConn3 -- T_152182710_330000;110000;35000;fixme_Жовтнева_330/RConn3 -- bus136/LConn1
  T_150153410_330000;150000;35000;6000_Прометей_330/RConn1 -- L_150153410/LConn1
  T_150153410_330000;150000;35000;6000_Прометей_330/RConn2 -- L_150153410/LConn2
  L_150153410/LConn3 -- T_150153410_330000;150000;35000;6000_Прометей_330/RConn3 -- bus137/LConn1
  T_165767625_750000;330000;15000_Дніпровська_750/RConn1 -- L_165767625/LConn1
  T_165767625_750000;330000;15000_Дніпровська_750/RConn2 -- L_165767625/LConn2
  L_165767625/LConn3 -- T_165767625_750000;330000;15000_Дніпровська_750/RConn3 -- bus138/LConn1
  T_228999814_330000;150000;35000_Молочанська_330/RConn1 -- L_228999814/LConn1
  T_228999814_330000;150000;35000_Молочанська_330/RConn2 -- L_228999814/LConn2
  L_228999814/LConn3 -- T_228999814_330000;150000;35000_Молочанська_330/RConn3 -- bus139/LConn1
  T_97343458_330000;220000;110000_Джанкой_330/RConn1 -- L_97343458/LConn1
  T_97343458_330000;220000;110000_Джанкой_330/RConn2 -- L_97343458/LConn2
  L_97343458/LConn3 -- T_97343458_330000;220000;110000_Джанкой_330/RConn3 -- bus140/LConn1
  T_100454075__/RConn1 -- L_100454075/LConn1
  T_100454075__/RConn2 -- L_100454075/LConn2
  L_100454075/LConn3 -- T_100454075__/RConn3 -- bus141/LConn1
  T_296062370_330000;150000;35000_Кварцит_330/RConn1 -- L_296062370/LConn1
  T_296062370_330000;150000;35000_Кварцит_330/RConn2 -- L_296062370/LConn2
  L_296062370/LConn3 -- T_296062370_330000;150000;35000_Кварцит_330/RConn3 -- bus142/LConn1
  T_202269421_330000;150000;10000_Українка_330/RConn1 -- L_202269421/LConn1
  T_202269421_330000;150000;10000_Українка_330/RConn2 -- L_202269421/LConn2
  L_202269421/LConn3 -- T_202269421_330000;150000;10000_Українка_330/RConn3 -- bus143/LConn1
  T_325748197__/RConn1 -- L_325748197/LConn1
  T_325748197__/RConn2 -- L_325748197/LConn2
  L_325748197/LConn3 -- T_325748197__/RConn3 -- bus144/LConn1
  T_107808612__/RConn1 -- L_107808612/LConn1
  T_107808612__/RConn2 -- L_107808612/LConn2
  L_107808612/LConn3 -- T_107808612__/RConn3 -- bus145/LConn1
  T_296062375_330000;150000;35000_Побузька_330/RConn1 -- L_296062375/LConn1
  T_296062375_330000;150000;35000_Побузька_330/RConn2 -- L_296062375/LConn2
  L_296062375/LConn3 -- T_296062375_330000;150000;35000_Побузька_330/RConn3 -- bus146/LConn1
  T_107811059_750000;330000_/RConn1 -- L_107811059/LConn1
  T_107811059_750000;330000_/RConn2 -- L_107811059/LConn2
  L_107811059/LConn3 -- T_107811059_750000;330000_/RConn3 -- bus147/LConn1
